simulink model "AmpelkreuzungV5_9"  (R2024b)
settings: Solver=FixedStepAuto  StartTime=0.0  StopTime=5000  FixedStep=1  RelTol=1e-3
model workspace (MATLAB code in the model file):
  | function [autos_l1, autos_rg1, autos_2l, autos_2rg, autos_3l, autos_3rg, autos_4, fehler] = generateCars(Auslastung)
  |     if (auslastung == 1)
  |         autos_l1 = round(randn());
  |         autos_rg1 = round(randn());
  |         autos_2l = round(randn());
  |         autos_2rg = round(randn());
  |         autos_3l = round(randn());
  |         autos_3rg = round(randn());
  |         autos_4 = round(randn());
  |     else
  |         fehler = 1;
  |     end
  | 
  |     if (auslastung == 2)
  |         autos_l1 = round(randn());
  |         autos_rg1 = round(4 + 2 * randn());
  |         autos_2l = round(1 + randn());
  |         autos_2rg = round(4 + 2 * randn());
  |         autos_3l = round(randn());
  |         autos_3rg = round(2 + randn());
  |         autos_4 = round(1 + randn());
  |     else
  |         fehler = 1;
  |     end
  | 
  |     if (auslastung == 3)
  |         autos_l1 = round(1.5 + randn());
  |         autos_rg1 = round(7 + 2 * randn());
  |         autos_2l = round(2 + randn());
  |         autos_2rg = round(7 + 2 * randn());
  |         autos_3l = round(2 * randn());
  |         autos_3rg = round(3 + randn());
  |         autos_4 = round(2 + randn());
  |     else
  |         fehler = 1;
  |     end
  | 
  |     if (auslastung == 4)
  |         autos_l1 = round(2.5 + randn());
  |         autos_rg1 = round(13 + 3 * randn());
  |         autos_2l = round(5 + randn());
  |         autos_2rg = round(13 + 3 * randn());
  |         autos_3l = round(2 + randn());
  |         autos_3rg = round(2 + randn());
  |         autos_4 = round(5 + randn());
  |     else
  |         fehler = 1;
  |     end
  | end
(part 2 of 3)

== stateflow chart AmpelkreuzungV5_9/Chart ==
  state Start
    entry:
    clear all;
    rot1_l = 1;
    gelb1_l = 0;
    gruen1_l = 0;
    rot1_rg = 1;
    gelb1_rg = 0;
    gruen1_rg = 0;
    rot2 = 1;
    gelb2 = 0;
    gruen2 = 0;
    rot3_l = 1;
    gelb3_l = 0;
    gruen3_l = 0;
    rot3_rg = 1;
    gelb3_rg = 0;
    gruen3_rg = 0;
    rot4 = 1;
    gelb4 = 0;
    gruen4 = 0;
    rot5 = 1;
    gruen5 = 0;
    rot6 = 1;
    gruen6 = 0;
    rot7 = 1;
    gruen7 = 0;
    rot8 = 1;
    gruen8 = 0;
    timeCounter = 0;
    timer_spuren = [0 0 0 0 0 0 0];
    gesamtZeit = 0;
    gesamte_autos = 0;
    %alle_autos = [0 0 0 0 0 0 0; 0 0 0 0 0 0 0];
    spur1 = zeros(1,N / 2);
    spur2 = zeros(1,N / 2);
    spur3 = zeros(1,N / 2);
    spur4 = zeros(1,N / 2);
    spur5 = zeros(1,N / 2);
    spur6 = zeros(1,N / 2);
    spur7 = zeros(1,N / 2);
    autos_auf_spur1 = 0;
    autos_auf_spur2 = 0;
    autos_auf_spur3 = 0;
    autos_auf_spur4 = 0;
    autos_auf_spur5 = 0;
    autos_auf_spur6 = 0;
    autos_auf_spur7 = 0;
    counter = [0 0 0 0 0 0 0];
    anz_autos1 = 0;
    anz_autos2 = 0;
    anz_autos3 = 0;
    anz_autos4 = 0;
    anz_autos5 = 0;
    anz_autos6 = 0;
    anz_autos7 = 0;
    wartezeit_spur1_ges = 0;
    wartezeit_spur2_ges = 0;
    wartezeit_spur3_ges = 0;
    wartezeit_spur4_ges = 0;
    wartezeit_spur5_ges = 0;
    wartezeit_spur6_ges = 0;
    wartezeit_spur7_ges = 0;
    krit1 = 0;
    krit2 = 0;
    krit3 = 0;
  state dokumentiere_startzeiten_initialisiere_wartezeiten
    en:
    startzeiten1 = spur1;
    startzeiten2 = spur2;
    startzeiten3 = spur3;
    startzeiten4 = spur4;
    startzeiten5 = spur5;
    startzeiten6 = spur6;
    startzeiten7 = spur7;
    wartezeiten1 = zeros(1, length(startzeiten1));
    wartezeiten2 = zeros(1, length(startzeiten2));
    wartezeiten3 = zeros(1, length(startzeiten3));
    wartezeiten4 = zeros(1, length(startzeiten4));
    wartezeiten5 = zeros(1, length(startzeiten5));
    wartezeiten6 = zeros(1, length(startzeiten6));
    wartezeiten7 = zeros(1, length(startzeiten7));
  state endzeiten_initialisieren
    en:
    endzeiten1 = zeros(1, length(spur1));
    endzeiten2 = zeros(1, length(spur2));
    endzeiten3 = zeros(1, length(spur3));
    endzeiten4 = zeros(1, length(spur4));
    endzeiten5 = zeros(1, length(spur5));
    endzeiten6 = zeros(1, length(spur6));
    endzeiten7 = zeros(1, length(spur7));
  state rg1_ampel2_rotgelb
    entry:
    gelb1_rg = 1;
    gelb2 = 1;
  state l1_rg1_rotgelb
    entry:
    gelb1_l = 1;
    gelb1_rg = 1;
  state rg1_ampel2_gruen
    entry:
    rot1_rg = 0;
    gelb1_rg = 0;
    gruen1_rg = 1;
    rot2 = 0;
    gelb2 = 0;
    gruen2 = 1;
    rot7 = 0;
    gruen7 = 1;
    rot8 = 0;
    gruen8 = 1;
  state l1_rg1_gruen
    entry:
    rot1_l = 0;
    gelb1_l = 0;
    gruen1_l = 1;
    rot1_rg = 0;
    gelb1_rg = 0;
    gruen1_rg = 1;
    rot7 = 0;
    gruen7 = 1;
  state rg1_ampel2_rotgelb1
    entry:
    gelb1_rg = 1;
    gelb2 = 1;
  state rg1_ampel2_rotgelb2
    entry:
    gelb1_rg = 1;
    gelb2 = 1;
  state l1_rg1_rotgelb1
    entry:
    gelb1_l = 1;
    gelb1_rg = 1;
  state l1_rg1_rotgelb2
    entry:
    gelb1_l = 1;
    gelb1_rg = 1;
  state l1_gelb
    entry:
    gelb1_l = 1;
    gruen1_l = 0;
  state rg1_ampel2_gruen1
    entry:
    rot1_rg = 0;
    gelb1_rg = 0;
    gruen1_rg = 1;
    rot2 = 0;
    gelb2 = 0;
    gruen2 = 1;
    rot7 = 0;
    gruen7 = 1;
    rot8 = 0;
    gruen8 = 1;
  state rg1_ampel2_gruen2
    entry:
    rot1_rg = 0;
    gelb1_rg = 0;
    gruen1_rg = 1;
    rot2 = 0;
    gelb2 = 0;
    gruen2 = 1;
    rot7 = 0;
    gruen7 = 1;
    rot8 = 0;
    gruen8 = 1;
  state l1_rg1_gruen1
    entry:
    rot1_l = 0;
    gelb1_l = 0;
    gruen1_l = 1;
    rot1_rg = 0;
    gelb1_rg = 0;
    gruen1_rg = 1;
    rot7 = 0;
    gruen7 = 1;
  state rg1_ampel2_rotgelb3
    entry:
    gelb1_rg = 1;
    gelb2 = 1;
  state l1_rg1_gruen2
    entry:
    rot1_l = 0;
    gelb1_l = 0;
    gruen1_l = 1;
    rot1_rg = 0;
    gelb1_rg = 0;
    gruen1_rg = 1;
    rot7 = 0;
    gruen7 = 1;
  state l1_rot
    entry:
    rot1_l = 1;
    gelb1_l = 0;
  state l1_rg1_rotgelb3
    entry:
    gelb1_l = 1;
    gelb1_rg = 1;
  state Fuss7_rot1
    entry:
    rot7 = 1;
    gruen7 = 0;
  state rg1_ampel2_gruen3
    entry:
    rot1_rg = 0;
    gelb1_rg = 0;
    gruen1_rg = 1;
    rot2 = 0;
    gelb2 = 0;
    gruen2 = 1;
    rot7 = 0;
    gruen7 = 1;
    rot8 = 0;
    gruen8 = 1;
  state l1_gelb1
    entry:
    gelb1_l = 1;
    gruen1_l = 0;
  state l1_gelb2
    entry:
    gelb1_l = 1;
    gruen1_l = 0;
  state l1_rg1_gruen3
    entry:
    rot1_l = 0;
    gelb1_l = 0;
    gruen1_l = 1;
    rot1_rg = 0;
    gelb1_rg = 0;
    gruen1_rg = 1;
    rot7 = 0;
    gruen7 = 1;
  state l1_rot1
    entry:
    rot1_l = 1;
    gelb1_l = 0;
  state rg1_gelb1
    entry:
    gelb1_rg = 1;
    gruen1_rg = 0;
  state l1_rot2
    entry:
    rot1_l = 1;
    gelb1_l = 0;
  state ampel2_rotgelb
    entry:
    gelb2 = 1;
  state l1_rot4
    entry:
    rot1_l = 1;
    gelb1_l = 0;
  state Fuss7_rot2
    entry:
    rot7 = 1;
    gruen7 = 0;
  state Fuss7_rot4
    entry:
    rot7 = 1;
    gruen7 = 0;
  state ampel2_fuss8_gruen
    rot2 = 0;
    gelb2 = 0;
    gruen2 = 1;
    rot8 = 0;
    gruen8 = 1;
  state l1_gelb3
    entry:
    gelb1_l = 1;
    gruen1_l = 0;
  state rg1_rot1
    entry:
    gelb1_rg = 0;
    rot1_rg = 1;
  state l1_rot3
    entry:
    rot1_l = 1;
    gelb1_l = 0;
  state rg1_gelb2
    entry:
    gelb1_rg = 1;
    gruen1_rg = 0;
  state l1_rot6
    entry:
    rot1_l = 1;
    gelb1_l = 0;
  state l1_rot5
    entry:
    rot1_l = 1;
    gelb1_l = 0;
  state rg1_gelb4
    entry:
    gelb1_rg = 1;
    gruen1_rg = 0;
  state Fuss7_rot6
    entry:
    rot7 = 1;
    gruen7 = 0;
  state ampel2_rotgelb1
    entry:
    gelb2 = 1;
  state ampel2_rotgelb2
    entry:
    gelb2 = 1;
  state ampel2_fuss8_gruen1
    rot2 = 0;
    gelb2 = 0;
    gruen2 = 1;
    rot8 = 0;
    gruen8 = 1;
  state Fuss7_rot
    entry:
    rot7 = 1;
    gruen7 = 0;
  state ampel2_fuss8_gruen2
    rot2 = 0;
    gelb2 = 0;
    gruen2 = 1;
    rot8 = 0;
    gruen8 = 1;
  state rg1_rot6
    entry:
    gelb1_rg = 0;
    rot1_rg = 1;
  state rg1_rot13
    entry:
    gelb1_rg = 0;
    rot1_rg = 1;
  state l1_rot7
    entry:
    rot1_l = 1;
    gelb1_l = 0;
  state rg1_gelb7
    entry:
    gelb1_rg = 1;
    gruen1_rg = 0;
  state rg1_gelb
    entry:
    gelb1_rg = 1;
    gruen1_rg = 0;
  state fuss7_rot
    entry:
    rot7 = 1;
    gruen7 = 0;
  state rg1_rot20
    entry:
    gelb1_rg = 0;
    rot1_rg = 1;
  state rg1_rot
    entry:
    gelb1_rg = 0;
    rot1_rg = 1;
  state Fuss7_rot3
    entry:
    rot7 = 1;
    gruen7 = 0;
  state Fuss7_rot5
    entry:
    rot7 = 1;
    gruen7 = 0;
  state rg1_rot5
    entry:
    gelb1_rg = 0;
    rot1_rg = 1;
  state ampel2_rotgelb3
    entry:
    gelb2 = 1;
  state rg1_gelb3
    entry:
    gelb1_rg = 1;
    gruen1_rg = 0;
  state rg1_gelb5
    entry:
    gelb1_rg = 1;
    gruen1_rg = 0;
  state ampel2_fuss8_gruen3
    rot2 = 0;
    gelb2 = 0;
    gruen2 = 1;
    rot8 = 0;
    gruen8 = 1;
  state rg1_rot7
    entry:
    gelb1_rg = 0;
    rot1_rg = 1;
  state rg1_rot14
    entry:
    gelb1_rg = 0;
    rot1_rg = 1;
  state rg1_rot4
    entry:
    gelb1_rg = 0;
    rot1_rg = 1;
  state rg1_gelb6
    entry:
    gelb1_rg = 1;
    gruen1_rg = 0;
  state rg1_rot11
    entry:
    gelb1_rg = 0;
    rot1_rg = 1;
  state fuss8_rot7
    entry:
    rot8 = 1;
    gruen8 = 0;
  state rg1_rot17
    entry:
    gelb1_rg = 0;
    rot1_rg = 1;
  state fuss8_rot11
    entry:
    rot8 = 1;
    gruen8 = 0;
  state rg1_rot9
    entry:
    gelb1_rg = 0;
    rot1_rg = 1;
  state rg1_rot12
    entry:
    gelb1_rg = 0;
    rot1_rg = 1;
  state fuss8_rot8
    entry:
    rot8 = 1;
    gruen8 = 0;
  state rg1_rot21
    entry:
    gelb1_rg = 0;
    rot1_rg = 1;
  state rg1_rot16
    entry:
    gelb1_rg = 0;
    rot1_rg = 1
  state fuss8_rot9
    entry:
    rot8 = 1;
    gruen8 = 0;
  state rg1_rot15
    entry:
    gelb1_rg = 0;
    rot1_rg = 1
  state fuss8_rot5
    entry:
    rot8 = 1;
    gruen8 = 0;
  state fuss8_rot4
    entry:
    rot8 = 1;
    gruen8 = 0;
  state rg1_rot19
    entry:
    gelb1_rg = 0;
    rot1_rg = 1
  state ampel2_gelb8
    entry:
    gelb2 = 1;
    gruen2 = 0;
  state rg1_rot3
    entry:
    gelb1_rg = 0;
    rot1_rg = 1
  state rg1_rot18
    entry:
    gelb1_rg = 0;
    rot1_rg = 1
  state ampel2_gelb6
    entry:
    gelb2 = 1;
    gruen2 = 0;
  state ampel2_gelb11
    entry:
    gelb2 = 1;
    gruen2 = 0;
  state ampel2_gelb7
    entry:
    gelb2 = 1;
    gruen2 = 0;
  state ampel2_gelb5
    entry:
    gelb2 = 1;
    gruen2 = 0;
  state rg1_rot2
    entry:
    gelb1_rg = 0;
    rot1_rg = 1
  state ampel2_gelb4
    entry:
    gelb2 = 1;
    gruen2 = 0;
  state fuss8_rot10
    entry:
    rot8 = 1;
    gruen8 = 0;
  state fuss8_rot12
    entry:
    rot8 = 1;
    gruen8 = 0;
  state fuss8_rot1
    entry:
    rot8 = 1;
    gruen8 = 0;
  state fuss8_rot
    entry:
    rot8 = 1;
    gruen8 = 0;
  state ampel2_rot12
    rot2 = 1;
    gelb2 = 0;
  state ampel2_gelb9
    entry:
    gelb2 = 1;
    gruen2 = 0;
  state ampel2_rot11
    rot2 = 1;
    gelb2 = 0;
  state ampel2_gelb10
    entry:
    gelb2 = 1;
    gruen2 = 0;
  state ampel2_gelb1
    entry:
    gelb2 = 1;
    gruen2 = 0;
  state rg1_rot8
    entry:
    gelb1_rg = 0;
    rot1_rg = 1
  state ampel2_gelb
    entry:
    gelb2 = 1;
    gruen2 = 0;
  state rg1_rot10
    entry:
    gelb1_rg = 0;
    rot1_rg = 1
  state ampel2_rot13
    rot2 = 1;
    gelb2 = 0;
  state fuss8_rot3
    entry:
    rot8 = 1;
    gruen8 = 0;
  state ampel2_rot9
    rot2 = 1;
    gelb2 = 0;
  state ampel2_rot19
    rot2 = 1;
    gelb2 = 0;
  state fuss8_rot2
    entry:
    rot8 = 1;
    gruen8 = 0;
  state ampel2_rot17
    rot2 = 1;
    gelb2 = 0;
  state ampel2_rot
    rot2 = 1;
    gelb2 = 0;
  state ampel2_gelb3
    entry:
    gelb2 = 1;
    gruen2 = 0;
  state ampel2_gelb2
    entry:
    gelb2 = 1;
    gruen2 = 0;
  state ampel2_rot21
    rot2 = 1;
    gelb2 = 0;
  state ampel2_rot20
    rot2 = 1;
    gelb2 = 0;
  state ampel2_rot1
    rot2 = 1;
    gelb2 = 0;
  state ampel2_rot5
    rot2 = 1;
    gelb2 = 0;
  state ampel2_rot14
    rot2 = 1;
    gelb2 = 0;
  state ampel2_rot10
    rot2 = 1;
    gelb2 = 0;
  state ampel2_rot6
    rot2 = 1;
    gelb2 = 0;
  state ampel2_rot15
    rot2 = 1;
    gelb2 = 0;
  state ampel2_rot8
    rot2 = 1;
    gelb2 = 0;
  state rg3_rotgelb7
    entry:
    gelb3_rg = 1;
  state rg3_rotgelb4
    entry:
    gelb3_rg = 1;
  state rg3_rotgelb8
    entry:
    gelb3_rg = 1;
  state rg3_rotgelb5
    entry:
    gelb3_rg = 1;
  state ampel2_rot16
    rot2 = 1;
    gelb2 = 0;
  state ampel2_rot22
    rot2 = 1;
    gelb2 = 0;
  state ampel2_rot18
    rot2 = 1;
    gelb2 = 0;
  state ampel2_rot2
    rot2 = 1;
    gelb2 = 0;
  state ampel2_rot23
    rot2 = 1;
    gelb2 = 0;
  state ampel2_rot3
    rot2 = 1;
    gelb2 = 0;
  state rg3_rotgelb10
    entry:
    gelb3_rg = 1;
  state rg3_rotgelb11
    entry:
    gelb3_rg = 1;
  state rg3_rotgelb12
    entry:
    gelb3_rg = 1;
  state rg3_rotgelb
    entry:
    gelb3_rg = 1;
  state rg3_rotgelb9
    entry:
    gelb3_rg = 1;
  state rg3_rotgelb1
    entry:
    gelb3_rg = 1;
  state ampel2_rot7
    rot2 = 1;
    gelb2 = 0;
  state ampel2_rot4
    rot2 = 1;
    gelb2 = 0;
  state rg3_rotgelb2
    entry:
    gelb3_rg = 1;
  state l3_rotgelb_rg3_fuss6_gruen
    entry:
    gelb3_l = 1;
    rot3_rg = 0;
    gelb3_rg = 0;
    gruen3_rg = 1;
    rot6 = 0;
    gruen6 = 1;
  state rg3_fuss6_gruen
    entry:
    rot3_rg = 0;
    gelb3_rg = 0;
    gruen3_rg = 1;
    rot6 = 0;
    gruen6 = 1;
  state rg3_rotgelb3
    entry:
    gelb3_rg = 1;
  state ampel4_rotgelb
    entry:
    gelb4 = 1;
  state rg3_rotgelb6
    entry:
    gelb3_rg = 1;
  state l3_gruen
    entry:
    rot3_l = 0;
    gelb3_l = 0;
    gruen3_l = 1;
  state l3_rotgelb_rg3_fuss6_gruen1
    entry:
    gelb3_l = 1;
    rot3_rg = 0;
    gelb3_rg = 0;
    gruen3_rg = 1;
    rot6 = 0;
    gruen6 = 1;
  state rg3_fuss6_gruen1
    entry:
    rot3_rg = 0;
    gelb3_rg = 0;
    gruen3_rg = 1;
    rot6 = 0;
    gruen6 = 1;
  state l3_rotgelb_rg3_fuss6_gruen2
    entry:
    gelb3_l = 1;
    rot3_rg = 0;
    gelb3_rg = 0;
    gruen3_rg = 1;
    rot6 = 0;
    gruen6 = 1;
  state rg3_fuss6_gruen2
    entry:
    rot3_rg = 0;
    gelb3_rg = 0;
    gruen3_rg = 1;
    rot6 = 0;
    gruen6 = 1;
  state l3_gelb
    entry:
    gelb3_l = 1;
    gruen3_l = 0;
  state ampel4_rotgelb1
    entry:
    gelb4 = 1;
  state ampel4_rotgelb2
    entry:
    gelb4 = 1;
  state l3_gruen1
    entry:
    rot3_l = 0;
    gelb3_l = 0;
    gruen3_l = 1;
  state ampel4_fuss5_gruen
    entry:
    rot4 = 0;
    gelb4 = 0;
    gruen4 = 1;
    rot5 = 0;
    gruen5 = 1;
  state l3_rotgelb_rg3_fuss6_gruen3
    entry:
    gelb3_l = 1;
    rot3_rg = 0;
    gelb3_rg = 0;
    gruen3_rg = 1;
    rot6 = 0;
    gruen6 = 1;
  state rg3_fuss6_gruen3
    entry:
    rot3_rg = 0;
    gelb3_rg = 0;
    gruen3_rg = 1;
    rot6 = 0;
    gruen6 = 1;
  state l3_gruen2
    entry:
    rot3_l = 0;
    gelb3_l = 0;
    gruen3_l = 1;
  state l3_fuss6_rot
    entry:
    rot3_l = 1;
    gelb3_l = 0;
    rot6 = 1;
    gruen6 = 0;
  state ampel4_rotgelb3
    entry:
    gelb4 = 1;
  state l3_gelb_fuss6_rot
    entry:
    gelb3_l = 1;
    gruen3_l = 0;
  state l3_gelb1
    entry:
    gelb3_l = 1;
    gruen3_l = 0;
  state l3_gruen3
    entry:
    rot3_l = 0;
    gelb3_l = 0;
    gruen3_l = 1;
  state ampel4_fuss5_gruen2
    entry:
    rot4 = 0;
    gelb4 = 0;
    gruen4 = 1;
    rot5 = 0;
    gruen5 = 1;
  state ampel4_fuss5_gruen4
    entry:
    rot4 = 0;
    gelb4 = 0;
    gruen4 = 1;
    rot5 = 0;
    gruen5 = 1;
  state fuss6_rot2
    entry:
    rot6 = 1;
    gruen6 = 0;
  state l3_fuss6_rot3
    entry:
    rot3_l = 1;
    gelb3_l = 0;
    rot6 = 1;
    gruen6 = 0;
  state l3_gelb2
    entry:
    gelb3_l = 1;
    gruen3_l = 0;
  state l3_fuss6_rot1
    entry:
    rot3_l = 1;
    gelb3_l = 0;
    rot6 = 1;
    gruen6 = 0;
  state l3_rot1
    entry:
    rot3_l = 1;
    gelb3_l = 0;
  state ampel4_fuss5_gruen6
    entry:
    rot4 = 0;
    gelb4 = 0;
    gruen4 = 1;
    rot5 = 0;
    gruen5 = 1;
  state fuss6_rot
    entry:
    rot6 = 1;
    gruen6 = 0;
  state fuss6_rot4
    entry:
    rot6 = 1;
    gruen6 = 0;
  state rg3_gelb1
    entry:
    gelb3_rg = 1;
    gruen3_rg = 0;
  state rg3_gelb
    entry:
    gelb3_rg = 1;
    gruen3_rg = 0;
  state l3_rot_rg3_gelb
    entry:
    rot3_l = 1;
    gelb3_l = 0;
    gelb3_rg = 1;
    gruen3_rg = 0;
  state l3_fuss6_rot2
    entry:
    rot3_l = 1;
    gelb3_l = 0;
    rot6 = 1;
    gruen6 = 0;
  state l3_rot
    entry:
    rot3_l = 1;
    gelb3_l = 0;
  state fuss6_rot1
    entry:
    rot6 = 1;
    gruen6 = 0;
  state fuss6_rot3
    entry:
    rot6 = 1;
    gruen6 = 0;
  state rg3_rot_ampel4_rotgelb
    entry:
    rot3_rg = 1;
    gelb3_rg = 0;
    gelb4 = 1;
  state rg3_gelb2
    entry:
    gelb3_rg = 1;
    gruen3_rg = 0;
  state rg3_gelb3
    entry:
    gelb3_rg = 1;
    gruen3_rg = 0;
  state rg3_gelb4
    entry:
    gelb3_rg = 1;
    gruen3_rg = 0;
  state rg3_gelb5
    entry:
    gelb3_rg = 1;
    gruen3_rg = 0;
  state rg3_fuss5_rot
    entry:
    rot3_rg = 1;
    gelb3_rg = 0;
    rot5 = 1;
    gruen5 = 0;
  state fuss6_rot5
    entry:
    rot6 = 1;
    gruen6 = 0;
  state l3_rot_rg3_gelb1
    entry:
    rot3_l = 1;
    gelb3_l = 0;
    gelb3_rg = 1;
    gruen3_rg = 0;
  state rg3_gelb6
    entry:
    gelb3_rg = 1;
    gruen3_rg = 0;
  state rg3_rot_ampel4_rotgelb2
    entry:
    rot3_rg = 1;
    gelb3_rg = 0;
    gelb4 = 1;
  state rg3_rot_ampel4_rotgelb4
    entry:
    rot3_rg = 1;
    gelb3_rg = 0;
    gelb4 = 1;
  state rg3_rot_ampel4_rotgelb1
    entry:
    rot3_rg = 1;
    gelb3_rg = 0;
    gelb4 = 1;
  state rg3_fuss5_rot2
    entry:
    rot3_rg = 1;
    gelb3_rg = 0;
    rot5 = 1;
    gruen5 = 0;
  state rg3_fuss5_rot5
    entry:
    rot3_rg = 1;
    gelb3_rg = 0;
    rot5 = 1;
    gruen5 = 0;
  state rg3_rot_ampel4_rotgelb6
    entry:
    rot3_rg = 1;
    gelb3_rg = 0;
    gelb4 = 1;
  state ampel4_fuss5_gruen1
    entry:
    rot4 = 0;
    gelb4 = 0;
    gruen4 = 1;
    rot5 = 0;
    gruen5 = 1;
  state rg3_fuss5_rot6
    entry:
    rot3_rg = 1;
    gelb3_rg = 0;
    rot5 = 1;
    gruen5 = 0;
  state rg3_rot_ampel4_rotgelb3
    entry:
    rot3_rg = 1;
    gelb3_rg = 0;
    gelb4 = 1;
  state rg3_rot_ampel4_rotgelb5
    entry:
    rot3_rg = 1;
    gelb3_rg = 0;
    gelb4 = 1;
  state fuss5_rot
    entry:
    rot5 = 1;
    gruen5 = 0;
  state ampel4_fuss5_gruen3
    entry:
    rot4 = 0;
    gelb4 = 0;
    gruen4 = 1;
    rot5 = 0;
    gruen5 = 1;
  state ampel4_fuss5_gruen5
    entry:
    rot4 = 0;
    gelb4 = 0;
    gruen4 = 1;
    rot5 = 0;
    gruen5 = 1;
  state rg3_rot_ampel4_rotgelb7
    entry:
    rot3_rg = 1;
    gelb3_rg = 0;
    gelb4 = 1;
  state rg3_fuss5_rot1
    entry:
    rot3_rg = 1;
    gelb3_rg = 0;
    rot5 = 1;
    gruen5 = 0;
  state ampel4_fuss5_gruen7
    entry:
    rot4 = 0;
    gelb4 = 0;
    gruen4 = 1;
    rot5 = 0;
    gruen5 = 1;
  state fuss5_rot1
    entry:
    rot5 = 1;
    gruen5 = 0;
  state fuss5_rot2
    entry:
    rot5 = 1;
    gruen5 = 0;
  state rg3_fuss5_rot3
    entry:
    rot3_rg = 1;
    gelb3_rg = 0;
    rot5 = 1;
    gruen5 = 0;
  state rg3_fuss5_rot4
    entry:
    rot3_rg = 1;
    gelb3_rg = 0;
    rot5 = 1;
    gruen5 = 0;
  state fuss5_rot3
    entry:
    rot5 = 1;
    gruen5 = 0;
  state ampel4_gelb
    entry:
    gelb4 = 1;
    gruen4 = 0;
  state rg3_fuss5_rot7
    entry:
    rot3_rg = 1;
    gelb3_rg = 0;
    rot5 = 1;
    gruen5 = 0;
  state ampel4_rot
    entry:
    rot4 = 1;
    gelb4 = 0;
  state ampel4_rot2
    entry:
    rot4 = 1;
    gelb4 = 0;
  state ampel4_gelb1
    entry:
    gelb4 = 1;
    gruen4 = 0;
  state ampel4_gelb2
    entry:
    gelb4 = 1;
    gruen4 = 0;
  state ampel4_rot3
    entry:
    rot4 = 1;
    gelb4 = 0;
  state ampel4_rot5
    entry:
    rot4 = 1;
    gelb4 = 0;
  state ampel4_gelb3
    entry:
    gelb4 = 1;
    gruen4 = 0;
  state ampel4_rot4
    entry:
    rot4 = 1;
    gelb4 = 0;
  state ampel4_rot6
    entry:
    rot4 = 1;
    gelb4 = 0;
  state ampel4_rot7
    entry:
    rot4 = 1;
    gelb4 = 0;
  state ampel4_rot8
    entry:
    rot4 = 1;
    gelb4 = 0;
  (default) -> Start
  Start -> (junction 796) : {zeit_abstand = zeit_abstand_aus_auslastung(auslastung);}
  (junction 796) -> (junction 748) : {alle_autos_neu  = generiere_autos_neu(N, zeit_abstand, auslastung);}
  (junction 748) -> dokumentiere_startzeiten_initialisiere_wartezeiten : {[spur1, spur2, spur3, spur4, spur5, spur6, spur7] = spuren_aus_autos(alle_autos_neu, N);}
  dokumentiere_startzeiten_initialisiere_wartezeiten -> endzeiten_initialisieren
  endzeiten_initialisieren -> (junction 248)
  (junction 181) -> (junction 248) : {timeCounter = resetTimer()}
  (junction 248) -> (junction 1426) [order 1] : [auslastung == 5]
  (junction 248) -> (junction 1428) [order 2]
  (junction 179) -> (junction 181)
  (junction 1426) -> (junction 1092) : {alte_counter = counter;}
  (junction 1428) -> (junction 1430) [order 1] : [auslastung == 4]
  (junction 1428) -> (junction 1840) [order 2]
  (junction 1430) -> (junction 1670) : {alte_counter = counter;}
  (junction 1840) -> (junction 1843) [order 1] : [auslastung == 3]
  (junction 1840) -> (junction 3331) [order 2]
  (junction 1843) -> (junction 2751) : {alte_counter = counter;}
  (junction 3331) -> (junction 3333) : [auslastung == 1 || auslastung == 2]
  (junction 3333) -> (junction 3239) : {alte_counter = counter;}
  (junction 1092) -> (junction 1075) : after(1,sec)
      | {timeCounter = refresher(timeCounter, 1);}
  (junction 1075) -> (junction 1077) : {timer_spuren = countOnwards(timer_spuren,1,[1 1 1 1 1 1 1]);}
      |
      | %Linksabbieger1
  (junction 1077) -> (junction 1076) : {[autos_auf_spur1, spur1] = autos_auf_spur_generieren(spur1, gesamtZeit + timeCounter + 2, autos_auf_spur1);}
  (junction 1076) -> (junction 1081) : {autos_spur1_flag = false;}
  (junction 1670) -> (junction 1696) : after(1,sec)
      | {timeCounter = refresher(timeCounter, 1);}
  (junction 2751) -> (junction 2752) : after(1,sec)
      | {timeCounter = refresher(timeCounter, 1);}
  (junction 1081) -> (junction 1085) [order 1] : [autos_auf_spur1 == 0]
  (junction 1696) -> (junction 1673) : {timer_spuren = countOnwards(timer_spuren,1,[1 1 1 1 1 1 1]);}
      |
      | %Linksabbieger1
  (junction 1081) -> (junction 1084) [order 2]
  (junction 1085) -> rg1_ampel2_rotgelb
  (junction 2752) -> (junction 2755) : {timer_spuren = countOnwards(timer_spuren,1,[1 1 1 1 1 1 1]);}
      |
      | %Linksabbieger1
  (junction 1084) -> (junction 1074) [order 1] : [autos_auf_spur1 > 0]
  (junction 1084) -> (junction 1111) [order 2]
  (junction 1074) -> l1_rg1_rotgelb : {autos_spur1_flag = true;}
  rg1_ampel2_rotgelb -> (junction 1097) : after(1,sec)
      | {timeCounter = refresher(timeCounter, 1);}
  (junction 1673) -> (junction 1668) : {[autos_auf_spur1, spur1] = autos_auf_spur_generieren(spur1, gesamtZeit + timeCounter + 2, autos_auf_spur1);}
  (junction 2755) -> (junction 2748) : {[autos_auf_spur1, spur1] = autos_auf_spur_generieren(spur1, gesamtZeit + timeCounter + 2, autos_auf_spur1);}
  (junction 1097) -> rg1_ampel2_gruen : {timer_spuren = countOnwards(timer_spuren,1,[1 1 1 1 1 1 1]);}
  l1_rg1_rotgelb -> (junction 1082) : after(1,sec)
      | {timeCounter = refresher(timeCounter, 1);}
  (junction 1082) -> l1_rg1_gruen : {timer_spuren = countOnwards(timer_spuren,1,[1 1 1 1 1 1 1]);}
  (junction 3239) -> (junction 3238) : after(1,sec)
      | {timeCounter = refresher(timeCounter, 1);}
  (junction 1668) -> (junction 1687) : {autos_spur1_flag = false;}
  (junction 2748) -> (junction 2753) : {autos_spur1_flag = false;}
  (junction 3238) -> (junction 3241) : {timer_spuren = countOnwards(timer_spuren,1,[1 1 1 1 1 1 1]);}
      |
      | %Linksabbieger1
  rg1_ampel2_gruen -> (junction 1080) : {[autos_auf_spur2, spur2] = autos_auf_spur_generieren(spur2, gesamtZeit + timeCounter, autos_auf_spur2);}
  (junction 1687) -> (junction 1688) [order 1] : [autos_auf_spur1 == 0]
  (junction 1687) -> (junction 1690) [order 2]
  (junction 1688) -> rg1_ampel2_rotgelb1
  (junction 3241) -> (junction 3240) : {[autos_auf_spur1, spur1] = autos_auf_spur_generieren(spur1, gesamtZeit + timeCounter + 2, autos_auf_spur1);}
  (junction 2753) -> (junction 2754) [order 1] : [autos_auf_spur1 == 0]
  (junction 2754) -> rg1_ampel2_rotgelb2
  (junction 2753) -> (junction 2740) [order 2]
  (junction 1080) -> (junction 1098) : {[autos_auf_spur3, spur3] = autos_auf_spur_generieren(spur3, gesamtZeit + timeCounter, autos_auf_spur3);}
  l1_rg1_gruen -> (junction 1083) : {[autos_auf_spur1, spur1] = autos_auf_spur_generieren(spur1, gesamtZeit + timeCounter, autos_auf_spur1);}
  (junction 1690) -> (junction 1697) [order 1] : [autos_auf_spur1 > 0]
  (junction 1690) -> (junction 1741) [order 2]
  (junction 1697) -> l1_rg1_rotgelb1 : {autos_spur1_flag = true;}
  rg1_ampel2_rotgelb1 -> (junction 1698) : after(1,sec)
      | {timeCounter = refresher(timeCounter, 1);}
  (junction 2740) -> (junction 2746) [order 1] : [autos_auf_spur1 > 0]
  (junction 2740) -> (junction 2786) [order 2]
  (junction 2746) -> l1_rg1_rotgelb2 : {autos_spur1_flag = true;}
  rg1_ampel2_rotgelb2 -> (junction 2747) : after(1,sec)
      | {timeCounter = refresher(timeCounter, 1);}
  (junction 1083) -> (junction 1078) : {[autos_auf_spur2, spur2] = autos_auf_spur_generieren(spur2, gesamtZeit + timeCounter, autos_auf_spur2);}
  (junction 1098) -> (junction 1086) : {[autos_auf_spur4, spur4] = autos_auf_spur_generieren(spur4, gesamtZeit + timeCounter, autos_auf_spur4);}
  (junction 1078) -> (junction 1073) : after(8,sec)
      | {timeCounter = refresher(timeCounter, 8);}
  (junction 1698) -> rg1_ampel2_gruen1 : {timer_spuren = countOnwards(timer_spuren,1,[1 1 1 1 1 1 1]);}
  (junction 2747) -> rg1_ampel2_gruen2 : {timer_spuren = countOnwards(timer_spuren,1,[1 1 1 1 1 1 1]);}
  l1_rg1_rotgelb1 -> (junction 1715) : after(1,sec)
      | {timeCounter = refresher(timeCounter, 1);}
  (junction 3240) -> (junction 3243) : {autos_spur1_flag = false;}
  (junction 1073) -> l1_gelb : {timer_spuren = countOnwards(timer_spuren,8,[0 0 1 1 1 1 1]);}
  (junction 1086) -> (junction 1087) : after(45,sec)
      | {timeCounter = refresher(timeCounter, 45);}
  l1_rg1_rotgelb2 -> (junction 2742) : after(1,sec)
      | {timeCounter = refresher(timeCounter, 1);}
  (junction 1715) -> l1_rg1_gruen1 : {timer_spuren = countOnwards(timer_spuren,1,[1 1 1 1 1 1 1]);}
  (junction 2742) -> l1_rg1_gruen2 : {timer_spuren = countOnwards(timer_spuren,1,[1 1 1 1 1 1 1]);}
  l1_gelb -> (junction 1093) : after(3,sec)
      | {timeCounter = refresher(timeCounter, 3);}
  (junction 1087) -> Fuss7_rot1 : {timer_spuren = countOnwards(timer_spuren,45,[1 0 0 0 1 1 1]);}
  (junction 1093) -> (junction 1079) : {[autos_auf_spur1, spur1] = autos_auf_spur_generieren(spur1, gesamtZeit + timeCounter, autos_auf_spur1);}
  (junction 3243) -> (junction 3249) [order 1] : [autos_auf_spur1 == 0]
  (junction 3243) -> (junction 3244) [order 2]
  (junction 3249) -> rg1_ampel2_rotgelb3
  (junction 1079) -> l1_rot : {timer_spuren = countOnwards(timer_spuren,3,[0 0 1 1 1 1 1]);}
  (junction 3244) -> (junction 3245) [order 1] : [autos_auf_spur1 > 0]
  rg1_ampel2_gruen1 -> (junction 1704) : {[autos_auf_spur2, spur2] = autos_auf_spur_generieren(spur2, gesamtZeit + timeCounter, autos_auf_spur2);}
  (junction 3244) -> (junction 3120) [order 2]
  (junction 3245) -> l1_rg1_rotgelb3 : {autos_spur1_flag = true;}
  rg1_ampel2_gruen2 -> (junction 2749) : {[autos_auf_spur2, spur2] = autos_auf_spur_generieren(spur2, gesamtZeit + timeCounter, autos_auf_spur2);}
  rg1_ampel2_rotgelb3 -> (junction 3246) : after(1,sec)
      | {timeCounter = refresher(timeCounter, 1);}
  l1_rot -> (junction 1095) : {[anz_autos1, autos_auf_spur1, counter(1), endzeiten1] = generiere_gruenphase(1, 11, autos_auf_spur1, counter(1),  (gesamtZeit + timeCounter - 11), endzeiten1, startzeiten1, auslastung, autos_spur1_flag);}
  (junction 1704) -> (junction 1722) : {[autos_auf_spur3, spur3] = autos_auf_spur_generieren(spur3, gesamtZeit + timeCounter, autos_auf_spur3);}
  (junction 2749) -> (junction 2743) : {[autos_auf_spur3, spur3] = autos_auf_spur_generieren(spur3, gesamtZeit + timeCounter, autos_auf_spur3);}
  l1_rg1_gruen1 -> (junction 1720) : {[autos_auf_spur1, spur1] = autos_auf_spur_generieren(spur1, gesamtZeit + timeCounter, autos_auf_spur1);}
  (junction 3246) -> rg1_ampel2_gruen3 : {timer_spuren = countOnwards(timer_spuren,1,[1 1 1 1 1 1 1]);}
  (junction 1095) -> (junction 1096) : {wartezeiten1 = berechne_wartezeiten(startzeiten1, endzeiten1, alte_counter(1), counter(1), wartezeiten1);}
  l1_rg1_gruen2 -> (junction 2741) : {[autos_auf_spur1, spur1] = autos_auf_spur_generieren(spur1, gesamtZeit + timeCounter, autos_auf_spur1);}
  l1_rg1_rotgelb3 -> (junction 3247) : after(1,sec)
      | {timeCounter = refresher(timeCounter, 1);}
  (junction 1720) -> (junction 1711) : {[autos_auf_spur2, spur2] = autos_auf_spur_generieren(spur2, gesamtZeit + timeCounter, autos_auf_spur2);}
  (junction 1722) -> (junction 1712) : {[autos_auf_spur4, spur4] = autos_auf_spur_generieren(spur4, gesamtZeit + timeCounter, autos_auf_spur4);}
  (junction 2741) -> (junction 2744) : {[autos_auf_spur2, spur2] = autos_auf_spur_generieren(spur2, gesamtZeit + timeCounter, autos_auf_spur2);}
  (junction 2743) -> (junction 2750) : {[autos_auf_spur4, spur4] = autos_auf_spur_generieren(spur4, gesamtZeit + timeCounter, autos_auf_spur4);}
  (junction 1096) -> (junction 1099) : {wartezeit_spur1_ges = gesamt_wartezeit_pro_spur(wartezeiten1, wartezeit_spur1_ges, alte_counter(1), counter(1));}
  Fuss7_rot1 -> (junction 1072) : after(2,sec)
      | {timeCounter = refresher(timeCounter, 2);}
  (junction 3247) -> l1_rg1_gruen3 : {timer_spuren = countOnwards(timer_spuren,1,[1 1 1 1 1 1 1]);}
  (junction 1711) -> (junction 1721) : after(8,sec)
      | {timeCounter = refresher(timeCounter, 8);}
  (junction 2744) -> (junction 2745) : after(8,sec)
      | {timeCounter = refresher(timeCounter, 8);}
  (junction 1099) -> (junction 1090) : {gesamtwartezeit = berechne_gesamtwartezeit(wartezeit_spur1_ges, wartezeit_spur2_ges, wartezeit_spur3_ges, wartezeit_spur4_ges, wartezeit_spur5_ges, wartezeit_spur6_ges, wartezeit_spur7_ges);}
  (junction 1721) -> l1_gelb1 : {timer_spuren = countOnwards(timer_spuren,8,[0 0 1 1 1 1 1]);}
  (junction 1712) -> (junction 1723) : after(35,sec)
      | {timeCounter = refresher(timeCounter, 35);}
  (junction 2750) -> (junction 2758) : after(20,sec)
      | {timeCounter = refresher(timeCounter, 20);}
  (junction 2745) -> l1_gelb2 : {timer_spuren = countOnwards(timer_spuren,8,[0 0 1 1 1 1 1]);}
  (junction 1072) -> rg1_gelb1 : {timer_spuren = countOnwards(timer_spuren,2,[1 0 0 0 1 1 1]);}
  (junction 1090) -> l1_rot1 : {gesamte_autos = berechne_gesamte_autos(counter(1), counter(2), counter(3), counter(4), counter(5), counter(6), counter(7));}
  l1_gelb1 -> (junction 1724) : after(3,sec)
      | {timeCounter = refresher(timeCounter, 3);}
  (junction 1723) -> Fuss7_rot2 : {timer_spuren = countOnwards(timer_spuren,35,[1 0 0 0 1 1 1]);}
  (junction 2758) -> Fuss7_rot4 : {timer_spuren = countOnwards(timer_spuren,20,[1 0 0 0 1 1 1]);}
  l1_gelb2 -> (junction 2756) : after(3,sec)
      | {timeCounter = refresher(timeCounter, 3);}
  rg1_ampel2_gruen3 -> (junction 3242) : {[autos_auf_spur2, spur2] = autos_auf_spur_generieren(spur2, gesamtZeit + timeCounter, autos_auf_spur2);}
  (junction 1724) -> (junction 1719) : {[autos_auf_spur1, spur1] = autos_auf_spur_generieren(spur1, gesamtZeit + timeCounter, autos_auf_spur1);}
  l1_rot1 -> (junction 1088) : after(3,sec)
      | {timeCounter = refresher(timeCounter, 3);}
  (junction 2756) -> (junction 2757) : {[autos_auf_spur1, spur1] = autos_auf_spur_generieren(spur1, gesamtZeit + timeCounter, autos_auf_spur1);}
  rg1_gelb1 -> (junction 1089) : after(3,sec)
      | {timeCounter = refresher(timeCounter, 3);}
  (junction 1088) -> ampel2_rotgelb : {timer_spuren = countOnwards(timer_spuren,3,[1 0 1 1 1 1 1]);}
  (junction 3242) -> (junction 3258) : {[autos_auf_spur3, spur3] = autos_auf_spur_generieren(spur3, gesamtZeit + timeCounter, autos_auf_spur3);}
  (junction 1719) -> l1_rot2 : {timer_spuren = countOnwards(timer_spuren,3,[0 0 1 1 1 1 1]);}
  l1_rg1_gruen3 -> (junction 3248) : {[autos_auf_spur1, spur1] = autos_auf_spur_generieren(spur1, gesamtZeit + timeCounter, autos_auf_spur1);}
  (junction 2757) -> l1_rot4 : {timer_spuren = countOnwards(timer_spuren,3,[0 0 1 1 1 1 1]);}
  (junction 3248) -> (junction 3259) : {[autos_auf_spur2, spur2] = autos_auf_spur_generieren(spur2, gesamtZeit + timeCounter, autos_auf_spur2);}
  (junction 1089) -> (junction 1094) : {[autos_auf_spur2, spur2] = autos_auf_spur_generieren(spur2, gesamtZeit + timeCounter, autos_auf_spur2);}
  (junction 3258) -> (junction 3264) : {[autos_auf_spur4, spur4] = autos_auf_spur_generieren(spur4, gesamtZeit + timeCounter, autos_auf_spur4);}
  l1_rot2 -> (junction 1725) : {[anz_autos1, autos_auf_spur1, counter(1), endzeiten1] = generiere_gruenphase(1, 11, autos_auf_spur1, counter(1),  (gesamtZeit + timeCounter - 11), endzeiten1, startzeiten1, auslastung, autos_spur1_flag);}
  ampel2_rotgelb -> (junction 1091) : after(1,sec)
      | {timeCounter = refresher(timeCounter, 1);}
  l1_rot4 -> (junction 2759) : {[anz_autos1, autos_auf_spur1, counter(1), endzeiten1] = generiere_gruenphase(1, 11, autos_auf_spur1, counter(1),  (gesamtZeit + timeCounter - 11), endzeiten1, startzeiten1, auslastung, autos_spur1_flag);}
  (junction 3259) -> (junction 3265) : after(3,sec)
      | {timeCounter = refresher(timeCounter, 3);}
  (junction 1091) -> ampel2_fuss8_gruen : {timer_spuren = countOnwards(timer_spuren,1,[1 0 1 1 1 1 1]);}
  (junction 1725) -> (junction 1708) : {wartezeiten1 = berechne_wartezeiten(startzeiten1, endzeiten1, alte_counter(1), counter(1), wartezeiten1);}
  (junction 1094) -> rg1_rot1 : {timer_spuren = countOnwards(timer_spuren,3,[1 0 0 0 1 1 1]);}
  (junction 3265) -> l1_gelb3 : {timer_spuren = countOnwards(timer_spuren,3,[0 0 1 1 1 1 1]);}
  (junction 3264) -> (junction 3267) : after(5,sec)
      | {timeCounter = refresher(timeCounter, 5);}
  (junction 2759) -> (junction 2760) : {wartezeiten1 = berechne_wartezeiten(startzeiten1, endzeiten1, alte_counter(1), counter(1), wartezeiten1);}
  (junction 1708) -> (junction 1731) : {wartezeit_spur1_ges = gesamt_wartezeit_pro_spur(wartezeiten1, wartezeit_spur1_ges, alte_counter(1), counter(1));}
  Fuss7_rot2 -> (junction 1726) : after(2,sec)
      | {timeCounter = refresher(timeCounter, 2);}
  Fuss7_rot4 -> (junction 2762) : after(2,sec)
      | {timeCounter = refresher(timeCounter, 2);}
  (junction 2760) -> (junction 2761) : {wartezeit_spur1_ges = gesamt_wartezeit_pro_spur(wartezeiten1, wartezeit_spur1_ges, alte_counter(1), counter(1));}
  l1_gelb3 -> (junction 3260) : after(3,sec)
      | {timeCounter = refresher(timeCounter, 3);}
  (junction 3267) -> Fuss7_rot6 : {timer_spuren = countOnwards(timer_spuren,5,[1 0 0 0 1 1 1]);}
  (junction 1731) -> (junction 1727) : {gesamtwartezeit = berechne_gesamtwartezeit(wartezeit_spur1_ges, wartezeit_spur2_ges, wartezeit_spur3_ges, wartezeit_spur4_ges, wartezeit_spur5_ges, wartezeit_spur6_ges, wartezeit_spur7_ges);}
  ampel2_fuss8_gruen -> (junction 1107) : {[autos_auf_spur3, spur3] = autos_auf_spur_generieren(spur3, gesamtZeit + timeCounter, autos_auf_spur3);}
  rg1_rot1 -> (junction 1124) : {[anz_autos2, autos_auf_spur2, counter(2), endzeiten2] = generiere_gruenphase(2, 50, autos_auf_spur2, counter(2),  (gesamtZeit + timeCounter - 50), endzeiten2, startzeiten2, auslastung, autos_spur1_flag);}
  (junction 2761) -> (junction 2765) : {gesamtwartezeit = berechne_gesamtwartezeit(wartezeit_spur1_ges, wartezeit_spur2_ges, wartezeit_spur3_ges, wartezeit_spur4_ges, wartezeit_spur5_ges, wartezeit_spur6_ges, wartezeit_spur7_ges);}
  (junction 3260) -> (junction 3250) : {[autos_auf_spur1, spur1] = autos_auf_spur_generieren(spur1, gesamtZeit + timeCounter, autos_auf_spur1);}
  (junction 1726) -> rg1_gelb2 : {timer_spuren = countOnwards(timer_spuren,2,[1 0 0 0 1 1 1]);}
  (junction 1727) -> l1_rot3 : {gesamte_autos = berechne_gesamte_autos(counter(1), counter(2), counter(3), counter(4), counter(5), counter(6), counter(7));}
  (junction 2762) -> rg1_gelb4 : {timer_spuren = countOnwards(timer_spuren,2,[1 0 0 0 1 1 1]);}
  (junction 2765) -> l1_rot5 : {gesamte_autos = berechne_gesamte_autos(counter(1), counter(2), counter(3), counter(4), counter(5), counter(6), counter(7));}
  (junction 1107) -> (junction 1128) : {[autos_auf_spur4, spur4] = autos_auf_spur_generieren(spur4, gesamtZeit + timeCounter, autos_auf_spur4);}
  (junction 3250) -> l1_rot6 : {timer_spuren = countOnwards(timer_spuren,3,[0 0 1 1 1 1 1]);}
  l1_rot3 -> (junction 1728) : after(3,sec)
      | {timeCounter = refresher(timeCounter, 3);}
  (junction 1128) -> (junction 1127) : after(45,sec)
      | {timeCounter = refresher(timeCounter,45);}
  rg1_gelb2 -> (junction 1732) : after(3,sec)
      | {timeCounter = refresher(timeCounter, 3);}
  l1_rot6 -> (junction 3263) : {[anz_autos1, autos_auf_spur1, counter(1), endzeiten1] = generiere_gruenphase(1, 6, autos_auf_spur1, counter(1),  (gesamtZeit + timeCounter - 6), endzeiten1, startzeiten1, auslastung, autos_spur1_flag);}
  l1_rot5 -> (junction 2763) : after(3,sec)
      | {timeCounter = refresher(timeCounter, 3);}
  (junction 1728) -> ampel2_rotgelb1 : {timer_spuren = countOnwards(timer_spuren,3,[1 0 1 1 1 1 1]);}
  rg1_gelb4 -> (junction 2764) : after(3,sec)
      | {timeCounter = refresher(timeCounter, 3);}
  (junction 1127) -> Fuss7_rot : {timer_spuren = countOnwards(timer_spuren,45,[1 0 0 0 1 1 1]);}
  (junction 2763) -> ampel2_rotgelb2 : {timer_spuren = countOnwards(timer_spuren,3,[1 0 1 1 1 1 1]);}
  (junction 3263) -> (junction 3252) : {wartezeiten1 = berechne_wartezeiten(startzeiten1, endzeiten1, alte_counter(1), counter(1), wartezeiten1);}
  (junction 1732) -> (junction 1706) : {[autos_auf_spur2, spur2] = autos_auf_spur_generieren(spur2, gesamtZeit + timeCounter, autos_auf_spur2);}
  ampel2_rotgelb1 -> (junction 1729) : after(1,sec)
      | {timeCounter = refresher(timeCounter, 1);}
  (junction 2764) -> (junction 2768) : {[autos_auf_spur2, spur2] = autos_auf_spur_generieren(spur2, gesamtZeit + timeCounter, autos_auf_spur2);}
  (junction 1124) -> (junction 1121) : {wartezeiten2 = berechne_wartezeiten(startzeiten2, endzeiten2, alte_counter(2), counter(2), wartezeiten2);}
  (junction 3252) -> (junction 3268) : {wartezeit_spur1_ges = gesamt_wartezeit_pro_spur(wartezeiten1, wartezeit_spur1_ges, alte_counter(1), counter(1));}
  Fuss7_rot6 -> (junction 3261) : after(2,sec)
      | {timeCounter = refresher(timeCounter, 2);}
  ampel2_rotgelb2 -> (junction 2766) : after(1,sec)
      | {timeCounter = refresher(timeCounter, 1);}
  (junction 1729) -> ampel2_fuss8_gruen1 : {timer_spuren = countOnwards(timer_spuren,1,[1 0 1 1 1 1 1]);}
  (junction 1706) -> rg1_rot6 : {timer_spuren = countOnwards(timer_spuren,3,[1 0 0 0 1 1 1]);}
  (junction 3268) -> (junction 3262) : {gesamtwartezeit = berechne_gesamtwartezeit(wartezeit_spur1_ges, wartezeit_spur2_ges, wartezeit_spur3_ges, wartezeit_spur4_ges, wartezeit_spur5_ges, wartezeit_spur6_ges, wartezeit_spur7_ges);}
  (junction 2766) -> ampel2_fuss8_gruen2 : {timer_spuren = countOnwards(timer_spuren,1,[1 0 1 1 1 1 1]);}
  (junction 2768) -> rg1_rot13 : {timer_spuren = countOnwards(timer_spuren,3,[1 0 0 0 1 1 1]);}
  (junction 3262) -> l1_rot7 : {gesamte_autos = berechne_gesamte_autos(counter(1), counter(2), counter(3), counter(4), counter(5), counter(6), counter(7));}
  (junction 3261) -> rg1_gelb7 : {timer_spuren = countOnwards(timer_spuren,2,[1 0 0 0 1 1 1]);}
  ampel2_fuss8_gruen1 -> (junction 1733) : {[autos_auf_spur3, spur3] = autos_auf_spur_generieren(spur3, gesamtZeit + timeCounter, autos_auf_spur3);}
  rg1_rot6 -> (junction 1709) : {[anz_autos2, autos_auf_spur2, counter(2), endzeiten2] = generiere_gruenphase(2, 40, autos_auf_spur2, counter(2),  (gesamtZeit + timeCounter - 40), endzeiten2, startzeiten2, auslastung, autos_spur1_flag);}
  Fuss7_rot -> (junction 1114) : after(2,sec)
      | {timeCounter = refresher(timeCounter, 2);}
  rg1_rot13 -> (junction 2771) : {[anz_autos2, autos_auf_spur2, counter(2), endzeiten2] = generiere_gruenphase(2, 25, autos_auf_spur2, counter(2),  (gesamtZeit + timeCounter - 25), endzeiten2, startzeiten2, auslastung, autos_spur1_flag);}
  (junction 1121) -> (junction 1105) : {wartezeit_spur2_ges = gesamt_wartezeit_pro_spur(wartezeiten2, wartezeit_spur2_ges, alte_counter(2), counter(2));}
  ampel2_fuss8_gruen2 -> (junction 2769) : {[autos_auf_spur3, spur3] = autos_auf_spur_generieren(spur3, gesamtZeit + timeCounter, autos_auf_spur3);}
  l1_rot7 -> (junction 3256) : after(3,sec)
      | {timeCounter = refresher(timeCounter, 3);}
  (junction 1114) -> rg1_gelb : {timer_spuren = countOnwards(timer_spuren,2,[1 0 0 0 1 1 1]);}
  rg1_gelb7 -> (junction 3269) : after(2,sec)
      | {timeCounter = refresher(timeCounter, 2);}
  (junction 1733) -> (junction 1707) : {[autos_auf_spur4, spur4] = autos_auf_spur_generieren(spur4, gesamtZeit + timeCounter, autos_auf_spur4);}
  (junction 2769) -> (junction 2767) : {[autos_auf_spur4, spur4] = autos_auf_spur_generieren(spur4, gesamtZeit + timeCounter, autos_auf_spur4);}
  (junction 3256) -> fuss7_rot : {timer_spuren = countOnwards(timer_spuren,3,[1 0 1 1 1 1 1]);}
  (junction 1105) -> (junction 1101) : {gesamtwartezeit = berechne_gesamtwartezeit(wartezeit_spur1_ges, wartezeit_spur2_ges, wartezeit_spur3_ges, wartezeit_spur4_ges, wartezeit_spur5_ges, wartezeit_spur6_ges, wartezeit_spur7_ges)}
  (junction 1707) -> (junction 1713) : after(35,sec)
      | {timeCounter = refresher(timeCounter, 35);}
  (junction 3269) -> (junction 3266) : {[autos_auf_spur2, spur2] = autos_auf_spur_generieren(spur2, gesamtZeit + timeCounter, autos_auf_spur2);}
  rg1_gelb -> (junction 1100) : after(3,sec)
      | {timeCounter = refresher(timeCounter, 3);}
  (junction 2767) -> (junction 2770) : after(10,sec)
      | {timeCounter = refresher(timeCounter, 10);}
  (junction 1713) -> Fuss7_rot3 : {timer_spuren = countOnwards(timer_spuren,35,[1 0 0 0 1 1 1]);}
  (junction 1100) -> (junction 1109) : {[autos_auf_spur2, spur2] = autos_auf_spur_generieren(spur2, gesamtZeit + timeCounter, autos_auf_spur2);}
  (junction 2770) -> Fuss7_rot5 : {timer_spuren = countOnwards(timer_spuren,10,[1 0 0 0 1 1 1]);}
  (junction 3266) -> rg1_rot20 : {timer_spuren = countOnwards(timer_spuren,2,[1 0 0 0 1 1 1]);}
  (junction 1109) -> rg1_rot : {timer_spuren = countOnwards(timer_spuren,3,[1 0 0 0 1 1 1]);}
  (junction 1101) -> rg1_rot5 : {gesamte_autos = berechne_gesamte_autos(counter(1), counter(2), counter(3), counter(4), counter(5), counter(6), counter(7))}
  (junction 1709) -> (junction 1705) : {wartezeiten2 = berechne_wartezeiten(startzeiten2, endzeiten2, alte_counter(2), counter(2), wartezeiten2);}
  (junction 2771) -> (junction 2772) : {wartezeiten2 = berechne_wartezeiten(startzeiten2, endzeiten2, alte_counter(2), counter(2), wartezeiten2);}
  fuss7_rot -> (junction 3253) : after(1,sec)
      | {timeCounter = refresher(timeCounter, 1);}
  rg1_rot20 -> (junction 3270) : {[anz_autos2, autos_auf_spur2, counter(2), endzeiten2] = generiere_gruenphase(2, 9, autos_auf_spur2, counter(2),  (gesamtZeit + timeCounter - 9), endzeiten2, startzeiten2, auslastung, autos_spur1_flag);}
  rg1_rot -> (junction 1125) : {[anz_autos2, autos_auf_spur2, counter(2), endzeiten2] = generiere_gruenphase(2, 65, autos_auf_spur2, counter(2),  (gesamtZeit + timeCounter - 65), endzeiten2, startzeiten2, auslastung, autos_spur1_flag);}
  (junction 3253) -> ampel2_rotgelb3 : {timer_spuren = countOnwards(timer_spuren,1,[1 0 1 1 1 1 1]);}
  Fuss7_rot3 -> (junction 1730) : after(2,sec)
      | {timeCounter = refresher(timeCounter, 2);}
  (junction 1125) -> (junction 1110) : {wartezeiten2 = berechne_wartezeiten(startzeiten2, endzeiten2, alte_counter(2), counter(2), wartezeiten2);}
  (junction 1705) -> (junction 1716) : {wartezeit_spur2_ges = gesamt_wartezeit_pro_spur(wartezeiten2, wartezeit_spur2_ges, alte_counter(2), counter(2));}
  Fuss7_rot5 -> (junction 2779) : after(2,sec)
      | {timeCounter = refresher(timeCounter, 2);}
  rg1_rot5 -> (junction 1122)
  (junction 2772) -> (junction 2781) : {wartezeit_spur2_ges = gesamt_wartezeit_pro_spur(wartezeiten2, wartezeit_spur2_ges, alte_counter(2), counter(2));}
  (junction 1730) -> rg1_gelb3 : {timer_spuren = countOnwards(timer_spuren,2,[1 0 0 0 1 1 1]);}
  ampel2_rotgelb3 -> (junction 3251) : after(1,sec)
      | {timeCounter = refresher(timeCounter, 1);}
  (junction 2779) -> rg1_gelb5 : {timer_spuren = countOnwards(timer_spuren,2,[1 0 0 0 1 1 1]);}
  (junction 1110) -> (junction 1119) : {wartezeit_spur2_ges = gesamt_wartezeit_pro_spur(wartezeiten2, wartezeit_spur2_ges, alte_counter(2), counter(2));}
  (junction 3251) -> ampel2_fuss8_gruen3 : {timer_spuren = countOnwards(timer_spuren,1,[1 0 1 1 1 1 1]);}
  (junction 1716) -> (junction 1735) : {gesamtwartezeit = berechne_gesamtwartezeit(wartezeit_spur1_ges, wartezeit_spur2_ges, wartezeit_spur3_ges, wartezeit_spur4_ges, wartezeit_spur5_ges, wartezeit_spur6_ges, wartezeit_spur7_ges)}
  (junction 2781) -> (junction 2775) : {gesamtwartezeit = berechne_gesamtwartezeit(wartezeit_spur1_ges, wartezeit_spur2_ges, wartezeit_spur3_ges, wartezeit_spur4_ges, wartezeit_spur5_ges, wartezeit_spur6_ges, wartezeit_spur7_ges)}
  rg1_gelb3 -> (junction 1717) : after(3,sec)
      | {timeCounter = refresher(timeCounter, 3);}
  (junction 3270) -> (junction 3255) : {wartezeiten2 = berechne_wartezeiten(startzeiten2, endzeiten2, alte_counter(2), counter(2), wartezeiten2);}
  rg1_gelb5 -> (junction 2780) : after(3,sec)
      | {timeCounter = refresher(timeCounter, 3);}
  (junction 1717) -> (junction 1734) : {[autos_auf_spur2, spur2] = autos_auf_spur_generieren(spur2, gesamtZeit + timeCounter, autos_auf_spur2);}
  (junction 1119) -> (junction 1104) : {gesamtwartezeit = berechne_gesamtwartezeit(wartezeit_spur1_ges, wartezeit_spur2_ges, wartezeit_spur3_ges, wartezeit_spur4_ges, wartezeit_spur5_ges, wartezeit_spur6_ges, wartezeit_spur7_ges)}
  (junction 2780) -> (junction 2776) : {[autos_auf_spur2, spur2] = autos_auf_spur_generieren(spur2, gesamtZeit + timeCounter, autos_auf_spur2);}
  (junction 1734) -> rg1_rot7 : {timer_spuren = countOnwards(timer_spuren,3,[1 0 0 0 1 1 1]);}
  (junction 1735) -> rg1_rot11 : {gesamte_autos = berechne_gesamte_autos(counter(1), counter(2), counter(3), counter(4), counter(5), counter(6), counter(7))}
  ampel2_fuss8_gruen3 -> (junction 3254) : {[autos_auf_spur3, spur3] = autos_auf_spur_generieren(spur3, gesamtZeit + timeCounter, autos_auf_spur3);}
  (junction 2775) -> fuss8_rot7 : {gesamte_autos = berechne_gesamte_autos(counter(1), counter(2), counter(3), counter(4), counter(5), counter(6), counter(7))}
  (junction 2776) -> rg1_rot14 : {timer_spuren = countOnwards(timer_spuren,3,[1 0 0 0 1 1 1]);}
  (junction 1104) -> rg1_rot4 : {gesamte_autos = berechne_gesamte_autos(counter(1), counter(2), counter(3), counter(4), counter(5), counter(6), counter(7))}
  (junction 3254) -> rg1_gelb6 : {[autos_auf_spur4, spur4] = autos_auf_spur_generieren(spur4, gesamtZeit + timeCounter, autos_auf_spur4);}
  rg1_rot7 -> (junction 1710) : {[anz_autos2, autos_auf_spur2, counter(2), endzeiten2] = generiere_gruenphase(2, 55, autos_auf_spur2, counter(2),  (gesamtZeit + timeCounter - 55), endzeiten2, startzeiten2, auslastung, autos_spur1_flag);}
  (junction 3255) -> (junction 3257) : {wartezeit_spur2_ges = gesamt_wartezeit_pro_spur(wartezeiten2, wartezeit_spur2_ges, alte_counter(2), counter(2));}
  rg1_rot14 -> (junction 2773) : {[anz_autos2, autos_auf_spur2, counter(2), endzeiten2] = generiere_gruenphase(2, 30, autos_auf_spur2, counter(2),  (gesamtZeit + timeCounter - 30), endzeiten2, startzeiten2, auslastung, autos_spur1_flag);}
  rg1_rot4 -> (junction 1113)
  (junction 1710) -> (junction 1714) : {wartezeiten2 = berechne_wartezeiten(startzeiten2, endzeiten2, alte_counter(2), counter(2), wartezeiten2);}
  rg1_gelb6 -> (junction 3271) : after(3,sec)
      | {timeCounter = refresher(timeCounter, 3);}
  (junction 2773) -> (junction 2777) : {wartezeiten2 = berechne_wartezeiten(startzeiten2, endzeiten2, alte_counter(2), counter(2), wartezeiten2);}
  rg1_rot11 -> (junction 1762)
  (junction 3257) -> (junction 3273) : {gesamtwartezeit = berechne_gesamtwartezeit(wartezeit_spur1_ges, wartezeit_spur2_ges, wartezeit_spur3_ges, wartezeit_spur4_ges, wartezeit_spur5_ges, wartezeit_spur6_ges, wartezeit_spur7_ges)}
  fuss8_rot7 -> (junction 2784)
  (junction 3271) -> (junction 3272) : {[autos_auf_spur2, spur2] = autos_auf_spur_generieren(spur2, gesamtZeit + timeCounter, autos_auf_spur2);}
  (junction 1714) -> (junction 1718) : {wartezeit_spur2_ges = gesamt_wartezeit_pro_spur(wartezeiten2, wartezeit_spur2_ges, alte_counter(2), counter(2));}
  (junction 3272) -> rg1_rot17 : {timer_spuren = countOnwards(timer_spuren,3,[1 0 0 0 1 1 1]);}
  (junction 2777) -> (junction 2778) : {wartezeit_spur2_ges = gesamt_wartezeit_pro_spur(wartezeiten2, wartezeit_spur2_ges, alte_counter(2), counter(2));}
  (junction 3273) -> fuss8_rot11 : {gesamte_autos = berechne_gesamte_autos(counter(1), counter(2), counter(3), counter(4), counter(5), counter(6), counter(7))}
  rg1_rot17 -> (junction 3104) : {[anz_autos2, autos_auf_spur2, counter(2), endzeiten2] = generiere_gruenphase(2, 13, autos_auf_spur2, counter(2),  (gesamtZeit + timeCounter - 13 ), endzeiten2, startzeiten2, auslastung, autos_spur1_flag);}
  (junction 1113) -> (junction 1111)
  (junction 1122) -> (junction 1113)
  (junction 1718) -> (junction 1757) : {gesamtwartezeit = berechne_gesamtwartezeit(wartezeit_spur1_ges, wartezeit_spur2_ges, wartezeit_spur3_ges, wartezeit_spur4_ges, wartezeit_spur5_ges, wartezeit_spur6_ges, wartezeit_spur7_ges)}
  (junction 1111) -> (junction 1112)
  (junction 2778) -> (junction 2774) : {gesamtwartezeit = berechne_gesamtwartezeit(wartezeit_spur1_ges, wartezeit_spur2_ges, wartezeit_spur3_ges, wartezeit_spur4_ges, wartezeit_spur5_ges, wartezeit_spur6_ges, wartezeit_spur7_ges)}
  (junction 3104) -> (junction 3101) : {wartezeiten2 = berechne_wartezeiten(startzeiten2, endzeiten2, alte_counter(2), counter(2), wartezeiten2);}
  (junction 1757) -> rg1_rot9 : {gesamte_autos = berechne_gesamte_autos(counter(1), counter(2), counter(3), counter(4), counter(5), counter(6), counter(7))}
  (junction 2774) -> rg1_rot12 : {gesamte_autos = berechne_gesamte_autos(counter(1), counter(2), counter(3), counter(4), counter(5), counter(6), counter(7))}
  (junction 3101) -> (junction 3094) : {wartezeit_spur2_ges = gesamt_wartezeit_pro_spur(wartezeiten2, wartezeit_spur2_ges, alte_counter(2), counter(2));}
  fuss8_rot11 -> (junction 3102) : after(2,sec)
      | {timeCounter = refresher(timeCounter, 1);}
  rg1_rot9 -> (junction 1764)
  rg1_rot12 -> (junction 2799)
  (junction 3102) -> (junction 3103) : {timer_spuren = countOnwards(timer_spuren,2,[1 1 0 0 1 1 1]);}
  (junction 3094) -> (junction 3096) : {gesamtwartezeit = berechne_gesamtwartezeit(wartezeit_spur1_ges, wartezeit_spur2_ges, wartezeit_spur3_ges, wartezeit_spur4_ges, wartezeit_spur5_ges, wartezeit_spur6_ges, wartezeit_spur7_ges)}
  (junction 3096) -> rg1_rot21 : {gesamte_autos = berechne_gesamte_autos(counter(1), counter(2), counter(3), counter(4), counter(5), counter(6), counter(7))}
  (junction 1764) -> (junction 1741)
  (junction 1762) -> (junction 1764)
  (junction 1741) -> (junction 1751)
  (junction 2784) -> fuss8_rot8 [order 1] : [autos_auf_spur3 <= 2]
  (junction 2784) -> (junction 2806) [order 2]
  (junction 2786) -> (junction 2659)
  (junction 2799) -> rg1_rot16 [order 1] : [autos_auf_spur3 <= 2]
  rg1_rot21 -> (junction 3095)
  (junction 2799) -> (junction 2801) [order 2]
  fuss8_rot8 -> (junction 2787) : %after(2,sec)
      | %{timeCounter = refresher(timeCounter, 2);}
  rg1_rot16 -> (junction 2785) : %after(10,sec)
      | %{timeCounter = refresher(timeCounter, 10);}
  (junction 2806) -> fuss8_rot9 [order 1] : [autos_auf_spur3 > 2]
  (junction 2806) -> (junction 2844) [order 2]
  (junction 2801) -> rg1_rot15 [order 1] : [autos_auf_spur3 > 2]
  (junction 2801) -> (junction 2677) [order 2]
  rg1_rot15 -> (junction 2797) : after(15,sec)
      | {timeCounter = refresher(timeCounter, 15);}
  fuss8_rot9 -> (junction 2800) : after(10,sec)
      | {timeCounter = refresher(timeCounter, 10);}
  (junction 2785) -> fuss8_rot5 : %{timer_spuren = countOnwards(timer_spuren,10,[1 1 0 0 1 1 1]);}
  (junction 2797) -> fuss8_rot4 : {timer_spuren = countOnwards(timer_spuren,15,[1 1 0 0 1 1 1]);}
  fuss8_rot5 -> (junction 2782) : after(2,sec)
      | {timeCounter = refresher(timeCounter, 2);}
  (junction 3095) -> rg1_rot19 [order 1] : [autos_auf_spur3 <= 2]
  (junction 3095) -> (junction 3097) [order 2]
  (junction 3103) -> ampel2_gelb8 [order 1] : [autos_auf_spur3 <= 2]
  (junction 2787) -> ampel2_gelb6 : %{timer_spuren = countOnwards(timer_spuren,2,[1 1 0 0 1 1 1]);}
  (junction 3103) -> (junction 3098) [order 2]
  fuss8_rot4 -> (junction 2802) : after(2,sec)
      | {timeCounter = refresher(timeCounter, 2);}
  rg1_rot19 -> (junction 3099) : after(3,sec)
      | {timeCounter = refresher(timeCounter, 3);}
  ampel2_gelb8 -> (junction 3118) : after(3,sec)
      | {timeCounter = refresher(timeCounter, 3);}
  (junction 2800) -> ampel2_gelb7 : {timer_spuren = countOnwards(timer_spuren,10,[1 1 0 0 1 1 1]);}
  (junction 2782) -> ampel2_gelb5 : {timer_spuren = countOnwards(timer_spuren,2,[1 1 0 0 1 1 1]);}
  (junction 1112) -> rg1_rot3 [order 1] : [autos_auf_spur3 <= 2]
  (junction 1112) -> (junction 1115) [order 2]
  (junction 2802) -> ampel2_gelb4 : {timer_spuren = countOnwards(timer_spuren,2,[1 1 0 0 1 1 1]);}
  (junction 3097) -> rg1_rot18 [order 1] : [autos_auf_spur3 > 2]
  (junction 3097) -> (junction 3176) [order 2]
  rg1_rot3 -> (junction 1120) : after(7,sec)
      | {timeCounter = refresher(timeCounter, 7);}
  (junction 3098) -> ampel2_gelb11 [order 1] : [autos_auf_spur3 > 2]
  rg1_rot18 -> (junction 3100) : after(3,sec)
      | {timeCounter = refresher(timeCounter, 3);}
  (junction 3098) -> (junction 3184) [order 2]
  ampel2_gelb6 -> (junction 2788) : %after(3,sec)
      | %{timeCounter = refresher(timeCounter, 3);}
  (junction 1115) -> rg1_rot2 [order 1] : [autos_auf_spur3 > 2]
  ampel2_gelb11 -> (junction 3117) : after(3,sec)
      | {timeCounter = refresher(timeCounter, 3);}
  (junction 1115) -> (junction 1138) [order 2]
  (junction 3099) -> fuss8_rot10 : {timer_spuren = countOnwards(timer_spuren,3,[1 1 0 0 1 1 1]);}
  ampel2_gelb7 -> (junction 2793) : after(3,sec)
      | {timeCounter = refresher(timeCounter, 3);}
  ampel2_gelb5 -> (junction 2789) : after(3,sec)
      | {timeCounter = refresher(timeCounter, 3);}
  rg1_rot2 -> (junction 1116) : after(20,sec)
      | {timeCounter = refresher(timeCounter, 20);}
  ampel2_gelb4 -> (junction 2791) : after(3,sec)
      | {timeCounter = refresher(timeCounter, 3);}
  (junction 2793) -> (junction 2803) : {timer_spuren = countOnwards(timer_spuren,3,[1 1 0 0 1 1 1]);}
  (junction 2788) -> (junction 2804) : %{timer_spuren = countOnwards(timer_spuren,3,[1 1 0 0 1 1 1]);}
  (junction 1120) -> fuss8_rot1 : {timer_spuren = countOnwards(timer_spuren,7,[1 1 0 0 1 1 1]);}
  (junction 2791) -> (junction 2798) : {timer_spuren = countOnwards(timer_spuren,3,[1 1 0 0 1 1 1]);}
  (junction 2789) -> (junction 2795) : {timer_spuren = countOnwards(timer_spuren,3,[1 1 0 0 1 1 1]);}
  (junction 3100) -> fuss8_rot12 : {timer_spuren = countOnwards(timer_spuren,3,[1 1 0 0 1 1 1]);}
  (junction 2803) -> (junction 2807) : {[autos_auf_spur3, spur3] = autos_auf_spur_generieren(spur3, gesamtZeit + timeCounter, autos_auf_spur3);}
  (junction 2804) -> (junction 2809) : {[autos_auf_spur3, spur3] = autos_auf_spur_generieren(spur3, gesamtZeit + timeCounter, autos_auf_spur3);}
  (junction 1116) -> fuss8_rot : {timer_spuren = countOnwards(timer_spuren,20,[1 1 0 0 1 1 1]);}
  (junction 2798) -> (junction 2810) : {[autos_auf_spur3, spur3] = autos_auf_spur_generieren(spur3, gesamtZeit + timeCounter, autos_auf_spur3);}
  (junction 2795) -> (junction 2790) : {[autos_auf_spur3, spur3] = autos_auf_spur_generieren(spur3, gesamtZeit + timeCounter, autos_auf_spur3);}
  fuss8_rot10 -> (junction 3127) : after(2,sec)
      | {timeCounter = refresher(timeCounter, 2);}
  (junction 2807) -> ampel2_rot12 : {[autos_auf_spur4, spur4] = autos_auf_spur_generieren(spur4, gesamtZeit + timeCounter, autos_auf_spur4);}
  fuss8_rot12 -> (junction 3107) : after(2,sec)
      | {timeCounter = refresher(timeCounter, 2);}
  fuss8_rot1 -> (junction 1106) : after(2,sec)
      | {timeCounter = refresher(timeCounter, 2);}
  (junction 2810) -> ampel2_rot11 : {[autos_auf_spur4, spur4] = autos_auf_spur_generieren(spur4, gesamtZeit + timeCounter, autos_auf_spur4);}
  (junction 3127) -> ampel2_gelb9 : {timer_spuren = countOnwards(timer_spuren,2,[1 1 0 0 1 1 1]);}
  (junction 2809) -> ampel2_rot13 : {[autos_auf_spur4, spur4] = autos_auf_spur_generieren(spur4, gesamtZeit + timeCounter, autos_auf_spur4);}
  (junction 3107) -> ampel2_gelb10 : {timer_spuren = countOnwards(timer_spuren,2,[1 1 0 0 1 1 1]);}
  fuss8_rot -> (junction 1108) : after(2,sec)
      | {timeCounter = refresher(timeCounter, 2);}
  (junction 2790) -> ampel2_rot9 : {[autos_auf_spur4, spur4] = autos_auf_spur_generieren(spur4, gesamtZeit + timeCounter, autos_auf_spur4);}
  (junction 1106) -> ampel2_gelb1 : {timer_spuren = countOnwards(timer_spuren,2,[1 1 0 0 1 1 1]);}
  (junction 1108) -> ampel2_gelb : {timer_spuren = countOnwards(timer_spuren,2,[1 1 0 0 1 1 1]);}
  ampel2_rot12 -> (junction 2783) : {[anz_autos3, autos_auf_spur3, counter(3), endzeiten3] = generiere_gruenphase(3, 40, autos_auf_spur3, counter(3),  (gesamtZeit + timeCounter - 40), endzeiten3, startzeiten3, auslastung, autos_spur1_flag)}
  ampel2_gelb9 -> (junction 3112) : after(3,sec)
      | {timeCounter = refresher(timeCounter, 3);}
  ampel2_rot11 -> (junction 2805) : {[anz_autos3, autos_auf_spur3, counter(3), endzeiten3] = generiere_gruenphase(3, 35, autos_auf_spur3, counter(3),  (gesamtZeit + timeCounter -  35), endzeiten3, startzeiten3, auslastung, autos_spur1_flag)}
  ampel2_gelb10 -> (junction 3124) : after(3,sec)
      | {timeCounter = refresher(timeCounter, 3);}
  (junction 1751) -> rg1_rot8 [order 1] : [autos_auf_spur3 <= 2]
  (junction 1751) -> (junction 1742) [order 2]
  ampel2_gelb1 -> (junction 1130) : after(3,sec)
      | {timeCounter = refresher(timeCounter, 3);}
  (junction 3124) -> (junction 3125) : {timer_spuren = countOnwards(timer_spuren,3,[1 1 0 0 1 1 1]);}
  (junction 3112) -> (junction 3113) : {timer_spuren = countOnwards(timer_spuren,3,[1 1 0 0 1 1 1]);}
  rg1_rot8 -> (junction 1744) : after(7,sec)
      | {timeCounter = refresher(timeCounter, 7);}
  ampel2_gelb -> (junction 1129) : after(3,sec)
      | {timeCounter = refresher(timeCounter, 3);}
  (junction 1742) -> rg1_rot10 [order 1] : [autos_auf_spur3 > 2]
  (junction 3117) -> (junction 3126) : {timer_spuren = countOnwards(timer_spuren,3,[1 1 0 0 1 1 1]);}
  (junction 3118) -> (junction 3114) : {timer_spuren = countOnwards(timer_spuren,3,[1 1 0 0 1 1 1]);}
  (junction 1742) -> (junction 1768) [order 2]
  (junction 1129) -> (junction 1126) : {timer_spuren = countOnwards(timer_spuren,3,[1 1 0 0 1 1 1]);}
  (junction 1130) -> (junction 1123) : {timer_spuren = countOnwards(timer_spuren,3,[1 1 0 0 1 1 1]);}
  rg1_rot10 -> (junction 1739) : after(20,sec)
      | {timeCounter = refresher(timeCounter, 20);}
  (junction 2783) -> (junction 2792) : {wartezeiten3 = berechne_wartezeiten(startzeiten3, endzeiten3, alte_counter(3), counter(3), wartezeiten3);}
  (junction 3125) -> (junction 3119) : {[autos_auf_spur3, spur3] = autos_auf_spur_generieren(spur3, gesamtZeit + timeCounter, autos_auf_spur3);}
  (junction 3113) -> (junction 3115) : {[autos_auf_spur3, spur3] = autos_auf_spur_generieren(spur3, gesamtZeit + timeCounter, autos_auf_spur3);}
  (junction 2805) -> (junction 2796) : {wartezeiten3 = berechne_wartezeiten(startzeiten3, endzeiten3, alte_counter(3), counter(3), wartezeiten3);}
  (junction 1744) -> fuss8_rot3 : {timer_spuren = countOnwards(timer_spuren,7,[1 1 0 0 1 1 1]);}
  (junction 3126) -> (junction 3106) : {[autos_auf_spur3, spur3] = autos_auf_spur_generieren(spur3, gesamtZeit + timeCounter, autos_auf_spur3);}
  (junction 3114) -> (junction 3111) : {[autos_auf_spur3, spur3] = autos_auf_spur_generieren(spur3, gesamtZeit + timeCounter, autos_auf_spur3);}
  (junction 1126) -> (junction 1117) : {[autos_auf_spur3, spur3] = autos_auf_spur_generieren(spur3, gesamtZeit + timeCounter, autos_auf_spur3);}
  (junction 1123) -> (junction 1118) : {[autos_auf_spur3, spur3] = autos_auf_spur_generieren(spur3, gesamtZeit + timeCounter, autos_auf_spur3);}
  (junction 3119) -> ampel2_rot19 : {[autos_auf_spur4, spur4] = autos_auf_spur_generieren(spur4, gesamtZeit + timeCounter, autos_auf_spur4);}
  (junction 3120) -> (junction 3108)
  (junction 2792) -> (junction 2794) : {wartezeit_spur3_ges = gesamt_wartezeit_pro_spur(wartezeiten3, wartezeit_spur3_ges, alte_counter(3), counter(3));}
  (junction 1739) -> fuss8_rot2 : {timer_spuren = countOnwards(timer_spuren,20,[1 1 0 0 1 1 1]);}
  (junction 3106) -> ampel2_rot17 : {[autos_auf_spur4, spur4] = autos_auf_spur_generieren(spur4, gesamtZeit + timeCounter, autos_auf_spur4);}
  (junction 3115) -> ampel2_rot21 : {[autos_auf_spur4, spur4] = autos_auf_spur_generieren(spur4, gesamtZeit + timeCounter, autos_auf_spur4);}
  (junction 2796) -> (junction 2820) : {wartezeit_spur3_ges = gesamt_wartezeit_pro_spur(wartezeiten3, wartezeit_spur3_ges, alte_counter(3), counter(3));}
  (junction 1117) -> ampel2_rot : {[autos_auf_spur4, spur4] = autos_auf_spur_generieren(spur4, gesamtZeit + timeCounter, autos_auf_spur4);}
  ampel2_rot13 -> (junction 2808) : {[anz_autos3, autos_auf_spur3, counter(3), endzeiten3] = generiere_gruenphase(3, 25, autos_auf_spur3, counter(3),  (gesamtZeit + timeCounter - 25), endzeiten3, startzeiten3, auslastung, autos_spur1_flag)}
  (junction 3111) -> ampel2_rot20 : {[autos_auf_spur4, spur4] = autos_auf_spur_generieren(spur4, gesamtZeit + timeCounter, autos_auf_spur4);}
  ampel2_rot9 -> (junction 2818) : {[anz_autos3, autos_auf_spur3, counter(3), endzeiten3] = generiere_gruenphase(3, 20, autos_auf_spur3, counter(3),  (gesamtZeit + timeCounter - 20), endzeiten3, startzeiten3, auslastung, autos_spur1_flag)}
  (junction 1118) -> ampel2_rot1 : {[autos_auf_spur4, spur4] = autos_auf_spur_generieren(spur4, gesamtZeit + timeCounter, autos_auf_spur4);}
  ampel2_rot19 -> (junction 3109) : {[anz_autos3, autos_auf_spur3, counter(3), endzeiten3] = generiere_gruenphase(3, 11, autos_auf_spur3, counter(3),  (gesamtZeit + timeCounter - 11), endzeiten3, startzeiten3, auslastung, autos_spur1_flag);}
  fuss8_rot3 -> (junction 1738) : after(2,sec)
      | {timeCounter = refresher(timeCounter, 2);}
  (junction 2794) -> (junction 2813) : {gesamtwartezeit = berechne_gesamtwartezeit(wartezeit_spur1_ges, wartezeit_spur2_ges, wartezeit_spur3_ges, wartezeit_spur4_ges, wartezeit_spur5_ges, wartezeit_spur6_ges, wartezeit_spur7_ges);}
  (junction 2808) -> (junction 2819) : {wartezeiten3 = berechne_wartezeiten(startzeiten3, endzeiten3, alte_counter(3), counter(3), wartezeiten3);}
  ampel2_rot17 -> (junction 3123) : {[anz_autos3, autos_auf_spur3, counter(3), endzeiten3] = generiere_gruenphase(3, 14, autos_auf_spur3, counter(3),  (gesamtZeit + timeCounter - 14), endzeiten3, startzeiten3, auslastung, autos_spur1_flag);}
  fuss8_rot2 -> (junction 1748) : after(2,sec)
      | {timeCounter = refresher(timeCounter, 2);}
  (junction 2820) -> (junction 2812) : {gesamtwartezeit = berechne_gesamtwartezeit(wartezeit_spur1_ges, wartezeit_spur2_ges, wartezeit_spur3_ges, wartezeit_spur4_ges, wartezeit_spur5_ges, wartezeit_spur6_ges, wartezeit_spur7_ges);}
  (junction 3108) -> (junction 3121)
  ampel2_rot -> (junction 1102) : {[anz_autos3, autos_auf_spur3, counter(3), endzeiten3] = generiere_gruenphase(3, 75, autos_auf_spur3, counter(3),  (gesamtZeit + timeCounter - 75), endzeiten3, startzeiten3, auslastung, autos_spur1_flag);}
  (junction 2818) -> (junction 2811) : {wartezeiten3 = berechne_wartezeiten(startzeiten3, endzeiten3, alte_counter(3), counter(3), wartezeiten3);}
  (junction 1738) -> ampel2_gelb3 : {timer_spuren = countOnwards(timer_spuren,2,[1 1 0 0 1 1 1]);}
  (junction 1748) -> ampel2_gelb2 : {timer_spuren = countOnwards(timer_spuren,2,[1 1 0 0 1 1 1]);}
  (junction 2813) -> (junction 2814) : {gesamte_autos = berechne_gesamte_autos(counter(1), counter(2), counter(3), counter(4), counter(5), counter(6), counter(7));}
  (junction 3121) -> (junction 3186)
  (junction 2812) -> (junction 2817) : {gesamte_autos = berechne_gesamte_autos(counter(1), counter(2), counter(3), counter(4), counter(5), counter(6), counter(7));}
  (junction 2819) -> (junction 2815) : {wartezeit_spur3_ges = gesamt_wartezeit_pro_spur(wartezeiten3, wartezeit_spur3_ges, alte_counter(3), counter(3));}
  (junction 3109) -> (junction 3122) : {wartezeiten3 = berechne_wartezeiten(startzeiten3, endzeiten3, alte_counter(3), counter(3), wartezeiten3);}
  (junction 2811) -> (junction 2816) : {wartezeit_spur3_ges = gesamt_wartezeit_pro_spur(wartezeiten3, wartezeit_spur3_ges, alte_counter(3), counter(3));}
  ampel2_gelb3 -> (junction 1765) : after(3,sec)
      | {timeCounter = refresher(timeCounter, 3);}
  ampel2_gelb2 -> (junction 1746) : after(3,sec)
      | {timeCounter = refresher(timeCounter, 3);}
  (junction 3123) -> (junction 3110) : {wartezeiten3 = berechne_wartezeiten(startzeiten3, endzeiten3, alte_counter(3), counter(3), wartezeiten3);}
  (junction 2814) -> (junction 2823) : {[anz_autos4, autos_auf_spur4, counter(4), endzeiten4] = generiere_gruenphase(4, 40, autos_auf_spur4, counter(4),  (gesamtZeit + timeCounter - 40), endzeiten4, startzeiten4, autos_spur1_flag)}
  (junction 1102) -> (junction 1131) : {wartezeiten3 = berechne_wartezeiten(startzeiten3, endzeiten3, alte_counter(3), counter(3), wartezeiten3);}
  (junction 2817) -> (junction 2824) : {[anz_autos4, autos_auf_spur4, counter(4), endzeiten4] = generiere_gruenphase(4, 35, autos_auf_spur4, counter(4),  (gesamtZeit + timeCounter - 35), endzeiten4, startzeiten4, autos_spur1_flag)}
  (junction 1746) -> (junction 1760) : {timer_spuren = countOnwards(timer_spuren,3,[1 1 0 0 1 1 1]);}
  (junction 1765) -> (junction 1758) : {timer_spuren = countOnwards(timer_spuren,3,[1 1 0 0 1 1 1]);}
  (junction 2815) -> (junction 2821) : {gesamtwartezeit = berechne_gesamtwartezeit(wartezeit_spur1_ges, wartezeit_spur2_ges, wartezeit_spur3_ges, wartezeit_spur4_ges, wartezeit_spur5_ges, wartezeit_spur6_ges, wartezeit_spur7_ges);}
  (junction 3122) -> (junction 3116) : {wartezeit_spur3_ges = gesamt_wartezeit_pro_spur(wartezeiten3, wartezeit_spur3_ges, alte_counter(3), counter(3));}
  (junction 2816) -> (junction 2825) : {gesamtwartezeit = berechne_gesamtwartezeit(wartezeit_spur1_ges, wartezeit_spur2_ges, wartezeit_spur3_ges, wartezeit_spur4_ges, wartezeit_spur5_ges, wartezeit_spur6_ges, wartezeit_spur7_ges)}
  (junction 2823) -> (junction 2822) : {wartezeiten4 = berechne_wartezeiten(startzeiten4, endzeiten4, alte_counter(4), counter(4), wartezeiten4);}
  (junction 3110) -> (junction 3147) : {wartezeit_spur3_ges = gesamt_wartezeit_pro_spur(wartezeiten3, wartezeit_spur3_ges, alte_counter(3), counter(3));}
  ampel2_rot21 -> (junction 3105) : {[anz_autos3, autos_auf_spur3, counter(3), endzeiten3] = generiere_gruenphase(3, 11, autos_auf_spur3, counter(3),  (gesamtZeit + timeCounter - 11), endzeiten3, startzeiten3, auslastung, autos_spur1_flag);}
  (junction 1131) -> (junction 1103) : {wartezeit_spur3_ges = gesamt_wartezeit_pro_spur(wartezeiten3, wartezeit_spur3_ges, alte_counter(3), counter(3));}
  (junction 2824) -> (junction 2828) : {wartezeiten4 = berechne_wartezeiten(startzeiten4, endzeiten4, alte_counter(4), counter(4), wartezeiten4);}
  (junction 1760) -> (junction 1753) : {[autos_auf_spur3, spur3] = autos_auf_spur_generieren(spur3, gesamtZeit + timeCounter, autos_auf_spur3);}
  (junction 1758) -> (junction 1743) : {[autos_auf_spur3, spur3] = autos_auf_spur_generieren(spur3, gesamtZeit + timeCounter, autos_auf_spur3);}
  ampel2_rot20 -> (junction 3153) : {[anz_autos3, autos_auf_spur3, counter(3), endzeiten3] = generiere_gruenphase(3, 14, autos_auf_spur3, counter(3),  (gesamtZeit + timeCounter - 14), endzeiten3, startzeiten3, auslastung, autos_spur1_flag);}
  (junction 2821) -> (junction 2826) : {gesamte_autos = berechne_gesamte_autos(counter(1), counter(2), counter(3), counter(4), counter(5), counter(6), counter(7));}
  ampel2_rot1 -> (junction 1158) : {[anz_autos3, autos_auf_spur3, counter(3), endzeiten3] = generiere_gruenphase(3, 62, autos_auf_spur3, counter(3),  (gesamtZeit + timeCounter - 62), endzeiten3, startzeiten3, auslastung, autos_spur1_flag);}
  (junction 2825) -> (junction 2827) : {gesamte_autos = berechne_gesamte_autos(counter(1), counter(2), counter(3), counter(4), counter(5), counter(6), counter(7));}
  (junction 3116) -> (junction 3136) : {gesamtwartezeit = berechne_gesamtwartezeit(wartezeit_spur1_ges, wartezeit_spur2_ges, wartezeit_spur3_ges, wartezeit_spur4_ges, wartezeit_spur5_ges, wartezeit_spur6_ges, wartezeit_spur7_ges);}
  (junction 3105) -> (junction 3139) : {wartezeiten3 = berechne_wartezeiten(startzeiten3, endzeiten3, alte_counter(3), counter(3), wartezeiten3);}
  (junction 2822) -> (junction 2831) : {wartezeit_spur4_ges = gesamt_wartezeit_pro_spur(wartezeiten4, wartezeit_spur4_ges, alte_counter(4), counter(4));}
  (junction 2826) -> (junction 2834) : {[anz_autos4, autos_auf_spur4, counter(4), endzeiten4] = generiere_gruenphase(4, 25, autos_auf_spur4, counter(4),  (gesamtZeit + timeCounter - 25), endzeiten4, startzeiten4, auslastung, autos_spur1_flag)}
  (junction 1753) -> ampel2_rot5 : {[autos_auf_spur4, spur4] = autos_auf_spur_generieren(spur4, gesamtZeit + timeCounter, autos_auf_spur4);}
  (junction 3147) -> (junction 3140) : {gesamtwartezeit = berechne_gesamtwartezeit(wartezeit_spur1_ges, wartezeit_spur2_ges, wartezeit_spur3_ges, wartezeit_spur4_ges, wartezeit_spur5_ges, wartezeit_spur6_ges, wartezeit_spur7_ges);}
  (junction 2828) -> (junction 2829) : {wartezeit_spur4_ges = gesamt_wartezeit_pro_spur(wartezeiten4, wartezeit_spur4_ges, alte_counter(4), counter(4));}
  (junction 2827) -> (junction 2830) : {[anz_autos4, autos_auf_spur4, counter(4), endzeiten4] = generiere_gruenphase(4, 20, autos_auf_spur4, counter(4),  (gesamtZeit + timeCounter - 20), endzeiten4, startzeiten4, auslastung, autos_spur1_flag);}
  (junction 1103) -> (junction 1143) : {gesamtwartezeit = berechne_gesamtwartezeit(wartezeit_spur1_ges, wartezeit_spur2_ges, wartezeit_spur3_ges, wartezeit_spur4_ges, wartezeit_spur5_ges, wartezeit_spur6_ges, wartezeit_spur7_ges);}
  (junction 3153) -> (junction 3156) : {wartezeiten3 = berechne_wartezeiten(startzeiten3, endzeiten3, alte_counter(3), counter(3), wartezeiten3);}
  (junction 1743) -> ampel2_rot6 : {[autos_auf_spur4, spur4] = autos_auf_spur_generieren(spur4, gesamtZeit + timeCounter, autos_auf_spur4);}
  (junction 1158) -> (junction 1153) : {wartezeiten3 = berechne_wartezeiten(startzeiten3, endzeiten3, alte_counter(3), counter(3), wartezeiten3);}
  (junction 2834) -> (junction 2832) : {wartezeiten4 = berechne_wartezeiten(startzeiten4, endzeiten4, alte_counter(4), counter(4), wartezeiten4);}
  (junction 3136) -> (junction 3152) : {gesamte_autos = berechne_gesamte_autos(counter(1), counter(2), counter(3), counter(4), counter(5), counter(6), counter(7));}
  (junction 2830) -> (junction 2833) : {wartezeiten4 = berechne_wartezeiten(startzeiten4, endzeiten4, alte_counter(4), counter(4), wartezeiten4);}
  (junction 3139) -> (junction 3142) : {wartezeit_spur3_ges = gesamt_wartezeit_pro_spur(wartezeiten3, wartezeit_spur3_ges, alte_counter(3), counter(3));}
  (junction 3140) -> (junction 3128) : {gesamte_autos = berechne_gesamte_autos(counter(1), counter(2), counter(3), counter(4), counter(5), counter(6), counter(7));}
  (junction 2831) -> (junction 2837) : {gesamtwartezeit = berechne_gesamtwartezeit(wartezeit_spur1_ges, wartezeit_spur2_ges, wartezeit_spur3_ges, wartezeit_spur4_ges, wartezeit_spur5_ges, wartezeit_spur6_ges, wartezeit_spur7_ges);}
  ampel2_rot5 -> (junction 1747) : {[anz_autos3, autos_auf_spur3, counter(3), endzeiten3] = generiere_gruenphase(3, 65, autos_auf_spur3, counter(3),  (gesamtZeit + timeCounter - 65), endzeiten3, startzeiten3, auslastung, autos_spur1_flag);}
  (junction 1143) -> (junction 1137) : {gesamte_autos = berechne_gesamte_autos(counter(1), counter(2), counter(3), counter(4), counter(5), counter(6), counter(7));}
  (junction 3156) -> (junction 3129) : {wartezeit_spur3_ges = gesamt_wartezeit_pro_spur(wartezeiten3, wartezeit_spur3_ges, alte_counter(3), counter(3));}
  (junction 2829) -> (junction 2838) : {gesamtwartezeit = berechne_gesamtwartezeit(wartezeit_spur1_ges, wartezeit_spur2_ges, wartezeit_spur3_ges, wartezeit_spur4_ges, wartezeit_spur5_ges, wartezeit_spur6_ges, wartezeit_spur7_ges);}
  (junction 2832) -> (junction 2841) : {wartezeit_spur4_ges = gesamt_wartezeit_pro_spur(wartezeiten4, wartezeit_spur4_ges, alte_counter(4), counter(4));}
  (junction 1153) -> (junction 1144) : {wartezeit_spur3_ges = gesamt_wartezeit_pro_spur(wartezeiten3, wartezeit_spur3_ges, alte_counter(3), counter(3));}
  (junction 3152) -> (junction 3131) : {[anz_autos4, autos_auf_spur4, counter(4), endzeiten4] = generiere_gruenphase(4, 55, autos_auf_spur4, counter(4),  (gesamtZeit + timeCounter -55), endzeiten4, startzeiten4, autos_spur1_flag);}
  (junction 2833) -> (junction 2839) : {wartezeit_spur4_ges = gesamt_wartezeit_pro_spur(wartezeiten4, wartezeit_spur4_ges, alte_counter(4), counter(4));}
  (junction 3128) -> (junction 3143) : {[anz_autos4, autos_auf_spur4, counter(4), endzeiten4] = generiere_gruenphase(4, 55, autos_auf_spur4, counter(4),  (gesamtZeit + timeCounter -55), endzeiten4, startzeiten4, autos_spur1_flag);}
  (junction 2837) -> ampel2_rot14 : {gesamte_autos = berechne_gesamte_autos(counter(1), counter(2), counter(3), counter(4), counter(5), counter(6), counter(7));}
  (junction 1137) -> (junction 1147) : {[anz_autos4, autos_auf_spur4, counter(4), endzeiten4] = generiere_gruenphase(4, 75, autos_auf_spur4, counter(4),  (gesamtZeit + timeCounter - 75), endzeiten4, startzeiten4, autos_spur1_flag);}
  (junction 3142) -> (junction 3145) : {gesamtwartezeit = berechne_gesamtwartezeit(wartezeit_spur1_ges, wartezeit_spur2_ges, wartezeit_spur3_ges, wartezeit_spur4_ges, wartezeit_spur5_ges, wartezeit_spur6_ges, wartezeit_spur7_ges);}
  (junction 2841) -> (junction 2840) : {gesamtwartezeit = berechne_gesamtwartezeit(wartezeit_spur1_ges, wartezeit_spur2_ges, wartezeit_spur3_ges, wartezeit_spur4_ges, wartezeit_spur5_ges, wartezeit_spur6_ges, wartezeit_spur7_ges);}
  (junction 2838) -> ampel2_rot10 : {gesamte_autos = berechne_gesamte_autos(counter(1), counter(2), counter(3), counter(4), counter(5), counter(6), counter(7));}
  (junction 3131) -> (junction 3154) : {wartezeiten4 = berechne_wartezeiten(startzeiten4, endzeiten4, alte_counter(4), counter(4), wartezeiten4);}
  (junction 3129) -> (junction 3155) : {gesamtwartezeit = berechne_gesamtwartezeit(wartezeit_spur1_ges, wartezeit_spur2_ges, wartezeit_spur3_ges, wartezeit_spur4_ges, wartezeit_spur5_ges, wartezeit_spur6_ges, wartezeit_spur7_ges);}
  (junction 2839) -> (junction 2842) : {gesamtwartezeit = berechne_gesamtwartezeit(wartezeit_spur1_ges, wartezeit_spur2_ges, wartezeit_spur3_ges, wartezeit_spur4_ges, wartezeit_spur5_ges, wartezeit_spur6_ges, wartezeit_spur7_ges);}
  (junction 1747) -> (junction 1759) : {wartezeiten3 = berechne_wartezeiten(startzeiten3, endzeiten3, alte_counter(3), counter(3), wartezeiten3);}
  (junction 1144) -> (junction 1156) : {gesamtwartezeit = berechne_gesamtwartezeit(wartezeit_spur1_ges, wartezeit_spur2_ges, wartezeit_spur3_ges, wartezeit_spur4_ges, wartezeit_spur5_ges, wartezeit_spur6_ges, wartezeit_spur7_ges);}
  (junction 3143) -> (junction 3132) : {wartezeiten4 = berechne_wartezeiten(startzeiten4, endzeiten4, alte_counter(4), counter(4), wartezeiten4);}
  (junction 1147) -> (junction 1146) : {wartezeiten4 = berechne_wartezeiten(startzeiten4, endzeiten4, alte_counter(4), counter(4), wartezeiten4);}
  (junction 2840) -> ampel2_rot15 : {gesamte_autos = berechne_gesamte_autos(counter(1), counter(2), counter(3), counter(4), counter(5), counter(6), counter(7));}
  (junction 3145) -> (junction 3157) : {gesamte_autos = berechne_gesamte_autos(counter(1), counter(2), counter(3), counter(4), counter(5), counter(6), counter(7));}
  (junction 2842) -> ampel2_rot8 : {gesamte_autos = berechne_gesamte_autos(counter(1), counter(2), counter(3), counter(4), counter(5), counter(6), counter(7));}
  (junction 3155) -> (junction 3146) : {gesamte_autos = berechne_gesamte_autos(counter(1), counter(2), counter(3), counter(4), counter(5), counter(6), counter(7));}
  (junction 3154) -> (junction 3144) : {wartezeit_spur4_ges = gesamt_wartezeit_pro_spur(wartezeiten4, wartezeit_spur4_ges, alte_counter(4), counter(4));}
  (junction 3157) -> (junction 3149) : {[anz_autos4, autos_auf_spur4, counter(4), endzeiten4] = generiere_gruenphase(4, 42, autos_auf_spur4, counter(4),  (gesamtZeit + timeCounter -42), endzeiten4, startzeiten4, auslastung, autos_spur1_flag);}
  (junction 1156) -> (junction 1148) : {gesamte_autos = berechne_gesamte_autos(counter(1), counter(2), counter(3), counter(4), counter(5), counter(6), counter(7));}
  (junction 1759) -> (junction 1756) : {wartezeit_spur3_ges = gesamt_wartezeit_pro_spur(wartezeiten3, wartezeit_spur3_ges, alte_counter(3), counter(3));}
  ampel2_rot14 -> (junction 2835) : after(1,sec)
      | {timeCounter = refresher(timeCounter, 1);}
  (junction 3132) -> (junction 3159) : {wartezeit_spur4_ges = gesamt_wartezeit_pro_spur(wartezeiten4, wartezeit_spur4_ges, alte_counter(4), counter(4));}
  (junction 3146) -> (junction 3148) : {[anz_autos4, autos_auf_spur4, counter(4), endzeiten4] = generiere_gruenphase(4, 42, autos_auf_spur4, counter(4),  (gesamtZeit + timeCounter -42), endzeiten4, startzeiten4, auslastung, autos_spur1_flag);}
  (junction 1146) -> (junction 1149) : {wartezeit_spur4_ges = gesamt_wartezeit_pro_spur(wartezeiten4, wartezeit_spur4_ges, alte_counter(4), counter(4));}
  (junction 1148) -> (junction 1155) : {[anz_autos4, autos_auf_spur4, counter(4), endzeiten4] = generiere_gruenphase(4, 62, autos_auf_spur4, counter(4),  (gesamtZeit + timeCounter - 62), endzeiten4, startzeiten4, auslastung, autos_spur1_flag);}
  ampel2_rot10 -> (junction 2836) : after(1,sec)
      | {timeCounter = refresher(timeCounter, 1);}
  ampel2_rot6 -> (junction 1737) : {[anz_autos3, autos_auf_spur3, counter(3), endzeiten3] = generiere_gruenphase(3, 52, autos_auf_spur3, counter(3),  (gesamtZeit + timeCounter - 52), endzeiten3, startzeiten3, auslastung, autos_spur1_flag);}
  (junction 3149) -> (junction 3133) : {wartezeiten4 = berechne_wartezeiten(startzeiten4, endzeiten4, alte_counter(4), counter(4), wartezeiten4);}
  ampel2_rot15 -> (junction 2846) : after(1,sec)
      | {timeCounter = refresher(timeCounter, 1);}
  (junction 2835) -> rg3_rotgelb7 : {timer_spuren = countOnwards(timer_spuren,1,[1 1 1 1 1 1 1]);}
  (junction 3148) -> (junction 3158) : {wartezeiten4 = berechne_wartezeiten(startzeiten4, endzeiten4, alte_counter(4), counter(4), wartezeiten4);}
  ampel2_rot8 -> (junction 2843) : after(1,sec)
      | {timeCounter = refresher(timeCounter, 1);}
  (junction 3144) -> (junction 3138) : {gesamtwartezeit = berechne_gesamtwartezeit(wartezeit_spur1_ges, wartezeit_spur2_ges, wartezeit_spur3_ges, wartezeit_spur4_ges, wartezeit_spur5_ges, wartezeit_spur6_ges, wartezeit_spur7_ges);}
  (junction 1155) -> (junction 1140) : {wartezeiten4 = berechne_wartezeiten(startzeiten4, endzeiten4, alte_counter(4), counter(4), wartezeiten4);}
  (junction 2836) -> rg3_rotgelb4 : {timer_spuren = countOnwards(timer_spuren,1,[1 1 1 1 1 1 1]);}
  (junction 1756) -> (junction 1740) : {gesamtwartezeit = berechne_gesamtwartezeit(wartezeit_spur1_ges, wartezeit_spur2_ges, wartezeit_spur3_ges, wartezeit_spur4_ges, wartezeit_spur5_ges, wartezeit_spur6_ges, wartezeit_spur7_ges);}
  (junction 2846) -> rg3_rotgelb8 : {timer_spuren = countOnwards(timer_spuren,1,[1 1 1 1 1 1 1]);}
  (junction 1737) -> (junction 1761) : {wartezeiten3 = berechne_wartezeiten(startzeiten3, endzeiten3, alte_counter(3), counter(3), wartezeiten3);}
  (junction 3159) -> (junction 3141) : {gesamtwartezeit = berechne_gesamtwartezeit(wartezeit_spur1_ges, wartezeit_spur2_ges, wartezeit_spur3_ges, wartezeit_spur4_ges, wartezeit_spur5_ges, wartezeit_spur6_ges, wartezeit_spur7_ges);}
  (junction 3133) -> (junction 3130) : {wartezeit_spur4_ges = gesamt_wartezeit_pro_spur(wartezeiten4, wartezeit_spur4_ges, alte_counter(4), counter(4));}
  (junction 2843) -> rg3_rotgelb5 : {timer_spuren = countOnwards(timer_spuren,1,[1 1 1 1 1 1 1]);}
  (junction 1149) -> (junction 1157) : {gesamtwartezeit = berechne_gesamtwartezeit(wartezeit_spur1_ges, wartezeit_spur2_ges, wartezeit_spur3_ges, wartezeit_spur4_ges, wartezeit_spur5_ges, wartezeit_spur6_ges, wartezeit_spur7_ges);}
  rg3_rotgelb7 -> (junction 2845)
  (junction 3158) -> (junction 3134) : {wartezeit_spur4_ges = gesamt_wartezeit_pro_spur(wartezeiten4, wartezeit_spur4_ges, alte_counter(4), counter(4));}
  rg3_rotgelb4 -> (junction 2655)
  (junction 1140) -> (junction 1136) : {wartezeit_spur4_ges = gesamt_wartezeit_pro_spur(wartezeiten4, wartezeit_spur4_ges, alte_counter(4), counter(4));}
  (junction 3138) -> ampel2_rot16 : {gesamte_autos = berechne_gesamte_autos(counter(1), counter(2), counter(3), counter(4), counter(5), counter(6), counter(7));}
  (junction 1740) -> (junction 1749) : {gesamte_autos = berechne_gesamte_autos(counter(1), counter(2), counter(3), counter(4), counter(5), counter(6), counter(7));}
  rg3_rotgelb8 -> (junction 2847)
  (junction 3130) -> (junction 3135) : {gesamtwartezeit = berechne_gesamtwartezeit(wartezeit_spur1_ges, wartezeit_spur2_ges, wartezeit_spur3_ges, wartezeit_spur4_ges, wartezeit_spur5_ges, wartezeit_spur6_ges, wartezeit_spur7_ges);}
  (junction 3141) -> ampel2_rot22 : {gesamte_autos = berechne_gesamte_autos(counter(1), counter(2), counter(3), counter(4), counter(5), counter(6), counter(7));}
  (junction 2845) -> (junction 2844)
  (junction 2847) -> (junction 2845)
  rg3_rotgelb5 -> (junction 2678)
  (junction 1761) -> (junction 1750) : {wartezeit_spur3_ges = gesamt_wartezeit_pro_spur(wartezeiten3, wartezeit_spur3_ges, alte_counter(3), counter(3));}
  (junction 2844) -> (junction 2673)
  (junction 1157) -> ampel2_rot2 : {gesamte_autos = berechne_gesamte_autos(counter(1), counter(2), counter(3), counter(4), counter(5), counter(6), counter(7));}
  (junction 3134) -> (junction 3150) : {gesamtwartezeit = berechne_gesamtwartezeit(wartezeit_spur1_ges, wartezeit_spur2_ges, wartezeit_spur3_ges, wartezeit_spur4_ges, wartezeit_spur5_ges, wartezeit_spur6_ges, wartezeit_spur7_ges);}
  (junction 2655) -> (junction 2677)
  (junction 2678) -> (junction 2655)
  (junction 2677) -> (junction 2656)
  (junction 1136) -> (junction 1141) : {gesamtwartezeit = berechne_gesamtwartezeit(wartezeit_spur1_ges, wartezeit_spur2_ges, wartezeit_spur3_ges, wartezeit_spur4_ges, wartezeit_spur5_ges, wartezeit_spur6_ges, wartezeit_spur7_ges);}
  (junction 3135) -> ampel2_rot18 : {gesamte_autos = berechne_gesamte_autos(counter(1), counter(2), counter(3), counter(4), counter(5), counter(6), counter(7));}
  (junction 1749) -> (junction 1752) : {[anz_autos4, autos_auf_spur4, counter(4), endzeiten4] = generiere_gruenphase(4, 65, autos_auf_spur4, counter(4),  (gesamtZeit + timeCounter - 65), endzeiten4, startzeiten4, autos_spur1_flag);}
  (junction 3150) -> ampel2_rot23 : {gesamte_autos = berechne_gesamte_autos(counter(1), counter(2), counter(3), counter(4), counter(5), counter(6), counter(7));}
  (junction 1141) -> ampel2_rot3 : {gesamte_autos = berechne_gesamte_autos(counter(1), counter(2), counter(3), counter(4), counter(5), counter(6), counter(7));}
  (junction 1750) -> (junction 1763) : {gesamtwartezeit = berechne_gesamtwartezeit(wartezeit_spur1_ges, wartezeit_spur2_ges, wartezeit_spur3_ges, wartezeit_spur4_ges, wartezeit_spur5_ges, wartezeit_spur6_ges, wartezeit_spur7_ges);}
  ampel2_rot16 -> (junction 3137) : after(1,sec)
      | {timeCounter = refresher(timeCounter, 1);}
  (junction 1752) -> (junction 1766) : {wartezeiten4 = berechne_wartezeiten(startzeiten4, endzeiten4, alte_counter(4), counter(4), wartezeiten4);}
  ampel2_rot22 -> (junction 3170) : after(1,sec)
      | {timeCounter = refresher(timeCounter, 1);}
  ampel2_rot18 -> (junction 3151) : after(1,sec)
      | {timeCounter = refresher(timeCounter, 1);}
  ampel2_rot2 -> (junction 1142) : after(1,sec)
      | {timeCounter = refresher(timeCounter, 1);}
  (junction 3137) -> rg3_rotgelb10 : {timer_spuren = countOnwards(timer_spuren,1,[1 1 1 1 1 1 1]);}
  (junction 1763) -> (junction 1745) : {gesamte_autos = berechne_gesamte_autos(counter(1), counter(2), counter(3), counter(4), counter(5), counter(6), counter(7));}
  ampel2_rot23 -> (junction 3174) : after(1,sec)
      | {timeCounter = refresher(timeCounter, 1);}
  ampel2_rot3 -> (junction 1163) : after(1,sec)
      | {timeCounter = refresher(timeCounter, 1);}
  (junction 3151) -> rg3_rotgelb12 : {timer_spuren = countOnwards(timer_spuren,1,[1 1 1 1 1 1 1]);}
  (junction 3170) -> rg3_rotgelb11 : {timer_spuren = countOnwards(timer_spuren,1,[1 1 1 1 1 1 1]);}
  (junction 1766) -> (junction 1754) : {wartezeit_spur4_ges = gesamt_wartezeit_pro_spur(wartezeiten4, wartezeit_spur4_ges, alte_counter(4), counter(4));}
  (junction 1745) -> (junction 1736) : {[anz_autos4, autos_auf_spur4, counter(4), endzeiten4] = generiere_gruenphase(4, 52, autos_auf_spur4, counter(4),  (gesamtZeit + timeCounter - 52), endzeiten4, startzeiten4, auslastung, autos_spur1_flag);}
  (junction 1142) -> rg3_rotgelb : {timer_spuren = countOnwards(timer_spuren,1,[1 1 1 1 1 1 1]);}
  (junction 3174) -> rg3_rotgelb9 : {timer_spuren = countOnwards(timer_spuren,1,[1 1 1 1 1 1 1]);}
  rg3_rotgelb10 -> (junction 3183)
  (junction 1163) -> rg3_rotgelb1 : {timer_spuren = countOnwards(timer_spuren,1,[1 1 1 1 1 1 1]);}
  (junction 2656) -> (junction 2659)
  (junction 2673) -> (junction 2656)
  rg3_rotgelb11 -> (junction 3172)
  (junction 2659) -> (junction 2660) : {[autos_auf_spur5, spur5] = autos_auf_spur_generieren(spur5, gesamtZeit + timeCounter, autos_auf_spur5);}
  (junction 1736) -> (junction 1755) : {wartezeiten4 = berechne_wartezeiten(startzeiten4, endzeiten4, alte_counter(4), counter(4), wartezeiten4);}
  rg3_rotgelb12 -> (junction 3171)
  rg3_rotgelb -> (junction 1133)
  (junction 3183) -> (junction 3176)
  (junction 3171) -> (junction 3183)
  (junction 3176) -> (junction 3161)
  rg3_rotgelb9 -> (junction 3175)
  (junction 1754) -> (junction 1777) : {gesamtwartezeit = berechne_gesamtwartezeit(wartezeit_spur1_ges, wartezeit_spur2_ges, wartezeit_spur3_ges, wartezeit_spur4_ges, wartezeit_spur5_ges, wartezeit_spur6_ges, wartezeit_spur7_ges);}
  rg3_rotgelb1 -> (junction 1150)
  (junction 3172) -> (junction 3184)
  (junction 3175) -> (junction 3172)
  (junction 3184) -> (junction 3166)
  (junction 1133) -> (junction 1138)
  (junction 1150) -> (junction 1133)
  (junction 1755) -> (junction 1769) : {wartezeit_spur4_ges = gesamt_wartezeit_pro_spur(wartezeiten4, wartezeit_spur4_ges, alte_counter(4), counter(4));}
  (junction 1138) -> (junction 1151) : {[autos_auf_spur5, spur5] = autos_auf_spur_generieren(spur5, gesamtZeit + timeCounter, autos_auf_spur5);}
  (junction 1777) -> ampel2_rot7 : {gesamte_autos = berechne_gesamte_autos(counter(1), counter(2), counter(3), counter(4), counter(5), counter(6), counter(7));}
  (junction 1769) -> (junction 1791) : {gesamtwartezeit = berechne_gesamtwartezeit(wartezeit_spur1_ges, wartezeit_spur2_ges, wartezeit_spur3_ges, wartezeit_spur4_ges, wartezeit_spur5_ges, wartezeit_spur6_ges, wartezeit_spur7_ges);}
  (junction 1791) -> ampel2_rot4 : {gesamte_autos = berechne_gesamte_autos(counter(1), counter(2), counter(3), counter(4), counter(5), counter(6), counter(7));}
  (junction 1151) -> (junction 1154) [order 1] : [autos_auf_spur5 == 0]
  (junction 1151) -> (junction 1139) [order 2]
  (junction 1154) -> (junction 1160) : after(1,sec)
      | {timeCounter = refresher(timeCounter, 1);}
  (junction 3161) -> (junction 3186)
  (junction 3166) -> (junction 3161)
  (junction 3186) -> (junction 3177) : {[autos_auf_spur5, spur5] = autos_auf_spur_generieren(spur5, gesamtZeit + timeCounter, autos_auf_spur5);}
  ampel2_rot7 -> (junction 1775) : after(1,sec)
      | {timeCounter = refresher(timeCounter, 1);}
  (junction 1139) -> (junction 1159) [order 1] : [autos_auf_spur5 > 0]
  (junction 1139) -> (junction 1184) [order 2]
  (junction 1159) -> l3_rotgelb_rg3_fuss6_gruen
  ampel2_rot4 -> (junction 1799) : after(1,sec)
      | {timeCounter = refresher(timeCounter, 1);}
  (junction 1775) -> rg3_rotgelb2 : {timer_spuren = countOnwards(timer_spuren,1,[1 1 1 1 1 1 1]);}
  (junction 1160) -> rg3_fuss6_gruen : {timer_spuren = countOnwards(timer_spuren,1,[1 1 1 1 1 1 1]);}
  (junction 1799) -> rg3_rotgelb3 : {timer_spuren = countOnwards(timer_spuren,1,[1 1 1 1 1 1 1]);}
  rg3_rotgelb2 -> (junction 1776)
  rg3_rotgelb3 -> (junction 1792)
  (junction 1776) -> (junction 1768)
  (junction 1792) -> (junction 1776)
  l3_rotgelb_rg3_fuss6_gruen -> (junction 1162) : {[autos_auf_spur6, spur6] = autos_auf_spur_generieren(spur6, gesamtZeit + timeCounter, autos_auf_spur6);}
  rg3_fuss6_gruen -> (junction 1132) : {[autos_auf_spur6, spur6] = autos_auf_spur_generieren(spur6, gesamtZeit + timeCounter, autos_auf_spur6);}
  (junction 1768) -> (junction 1783) : {[autos_auf_spur5, spur5] = autos_auf_spur_generieren(spur5, gesamtZeit + timeCounter, autos_auf_spur5);}
  (junction 1132) -> (junction 1161) : after(4,sec)
      | {timeCounter = refresher(timeCounter, 4);}
  (junction 1162) -> (junction 1152) : after(1,sec)
      | {timeCounter = refresher(timeCounter, 1);}
  (junction 1152) -> l3_gruen : {timer_spuren = countOnwards(timer_spuren,1,[1 1 1 1 1 0 1]);}
  (junction 1161) -> ampel4_rotgelb : {timer_spuren = countOnwards(timer_spuren,4,[1 1 1 1 1 0 1]);}
  (junction 1783) -> (junction 1770) [order 1] : [autos_auf_spur5 == 0]
  (junction 1783) -> (junction 1797) [order 2]
  (junction 1770) -> (junction 1767) : after(1,sec)
      | {timeCounter = refresher(timeCounter, 1);}
  (junction 2660) -> rg3_rotgelb6 [order 1] : [autos_auf_spur5 == 0]
  (junction 2660) -> (junction 2671) [order 2]
  ampel4_rotgelb -> (junction 1134) : after(1,sec)
      | {timeCounter = refresher(timeCounter, 1);}
  rg3_rotgelb6 -> (junction 2668) : after(1,sec)
      | {timeCounter = refresher(timeCounter, 1);}
  (junction 1797) -> (junction 1793) [order 1] : [autos_auf_spur5 > 0]
  (junction 1797) -> (junction 1800) [order 2]
  (junction 1793) -> l3_rotgelb_rg3_fuss6_gruen1
  (junction 2671) -> (junction 2667) [order 1] : [autos_auf_spur5 > 0]
  (junction 2671) -> (junction 2470) [order 2]
  l3_gruen -> (junction 1135) : after(8,sec)
      | {timeCounter = refresher(timeCounter, 8);}
  (junction 2667) -> l3_rotgelb_rg3_fuss6_gruen2
  (junction 1767) -> rg3_fuss6_gruen1 : {timer_spuren = countOnwards(timer_spuren,1,[1 1 1 1 1 1 1]);}
  (junction 2668) -> rg3_fuss6_gruen2 : {timer_spuren = countOnwards(timer_spuren,1,[1 1 1 1 1 1 1]);}
  (junction 1134) -> ampel4_fuss5_gruen : {timer_spuren = countOnwards(timer_spuren,1,[1 1 1 1 1 0 1]);}
  (junction 1135) -> l3_gelb : {timer_spuren = countOnwards(timer_spuren,8,[1 1 1 1 0 0 1]);}
  l3_rotgelb_rg3_fuss6_gruen1 -> (junction 1794) : {[autos_auf_spur6, spur6] = autos_auf_spur_generieren(spur6, gesamtZeit + timeCounter, autos_auf_spur6);}
  rg3_fuss6_gruen1 -> (junction 1771) : {[autos_auf_spur6, spur6] = autos_auf_spur_generieren(spur6, gesamtZeit + timeCounter, autos_auf_spur6);}
  l3_rotgelb_rg3_fuss6_gruen2 -> (junction 2674) : {[autos_auf_spur6, spur6] = autos_auf_spur_generieren(spur6, gesamtZeit + timeCounter, autos_auf_spur6);}
  rg3_fuss6_gruen2 -> (junction 2676) : {[autos_auf_spur6, spur6] = autos_auf_spur_generieren(spur6, gesamtZeit + timeCounter, autos_auf_spur6);}
  (junction 1771) -> (junction 1784) : after(4,sec)
      | {timeCounter = refresher(timeCounter, 4);}
  (junction 1794) -> (junction 1786) : after(1,sec)
      | {timeCounter = refresher(timeCounter, 1);}
  (junction 3177) -> (junction 3182) [order 1] : [autos_auf_spur5 == 0]
  (junction 2676) -> (junction 2658) : after(4,sec)
      | {timeCounter = refresher(timeCounter, 4);}
  (junction 3177) -> (junction 3173) [order 2]
  (junction 3182) -> (junction 3178) : after(1,sec)
      | {timeCounter = refresher(timeCounter, 1);}
  (junction 2674) -> (junction 2661) : after(1,sec)
      | {timeCounter = refresher(timeCounter, 1);}
  (junction 1786) -> l3_gruen1 : {timer_spuren = countOnwards(timer_spuren,1,[1 1 1 1 1 0 1]);}
  (junction 1784) -> ampel4_rotgelb1 : {timer_spuren = countOnwards(timer_spuren,4,[1 1 1 1 1 0 1]);}
  (junction 3173) -> (junction 3187) [order 1] : [autos_auf_spur5 > 0]
  (junction 3173) -> (junction 3203) [order 2]
  (junction 3187) -> l3_rotgelb_rg3_fuss6_gruen3
  l3_gelb -> (junction 1145) : after(3,sec)
      | {timeCounter = refresher(timeCounter, 3);}
  (junction 2661) -> l3_gruen2 : {timer_spuren = countOnwards(timer_spuren,1,[1 1 1 1 1 0 1]);}
  (junction 2658) -> ampel4_rotgelb2 : {timer_spuren = countOnwards(timer_spuren,4,[1 1 1 1 1 0 1]);}
  (junction 3178) -> rg3_fuss6_gruen3 : {timer_spuren = countOnwards(timer_spuren,1,[1 1 1 1 1 1 1]);}
  (junction 1145) -> (junction 1172) : {timer_spuren = countOnwards(timer_spuren,3,[1 1 1 1 0 0 1]);}
  ampel4_rotgelb1 -> (junction 1787) : after(1,sec)
      | {timeCounter = refresher(timeCounter, 1);}
  ampel4_rotgelb2 -> (junction 2675) : after(1,sec)
      | {timeCounter = refresher(timeCounter, 1);}
  l3_gruen1 -> (junction 1795) : after(8,sec)
      | {timeCounter = refresher(timeCounter, 8);}
  (junction 1172) -> l3_fuss6_rot : {[autos_auf_spur5, spur5] = autos_auf_spur_generieren(spur5, gesamtZeit + timeCounter, autos_auf_spur5);}
  l3_gruen2 -> (junction 2657) : after(6,sec)
      | {timeCounter = refresher(timeCounter, 6);}
  ampel4_fuss5_gruen -> (junction 1190) : {[autos_auf_spur7, spur7] = autos_auf_spur_generieren(spur7, gesamtZeit + timeCounter, autos_auf_spur7);}
  l3_rotgelb_rg3_fuss6_gruen3 -> (junction 3160) : {[autos_auf_spur6, spur6] = autos_auf_spur_generieren(spur6, gesamtZeit + timeCounter, autos_auf_spur6);}
  rg3_fuss6_gruen3 -> (junction 3167) : {[autos_auf_spur6, spur6] = autos_auf_spur_generieren(spur6, gesamtZeit + timeCounter, autos_auf_spur6);}
  (junction 1787) -> ampel4_fuss5_gruen2 : {timer_spuren = countOnwards(timer_spuren,1,[1 1 1 1 1 0 1]);}
  (junction 1190) -> (junction 1176) : after(6,sec)
      | {timeCounter = refresher(timeCounter, 6);}
  (junction 3167) -> (junction 3168) : after(4,sec)
      | {timeCounter = refresher(timeCounter, 4);}
  (junction 2675) -> ampel4_fuss5_gruen4 : {timer_spuren = countOnwards(timer_spuren,1,[1 1 1 1 1 0 1]);}
  (junction 1795) -> l3_gelb1 : {timer_spuren = countOnwards(timer_spuren,8,[1 1 1 1 0 0 1]);}
  (junction 3160) -> (junction 3162) : after(1,sec)
      | {timeCounter = refresher(timeCounter, 1);}
  (junction 2657) -> l3_gelb_fuss6_rot : {timer_spuren = countOnwards(timer_spuren,6,[1 1 1 1 0 0 1]);}
  l3_fuss6_rot -> (junction 1171) : {[anz_autos5, autos_auf_spur5, counter(5), endzeiten5] = generiere_gruenphase(5, 11, autos_auf_spur5, counter(5),  (gesamtZeit + timeCounter -11), endzeiten5, startzeiten5, auslastung, autos_spur1_flag);}
  (junction 3162) -> l3_gruen3 : {timer_spuren = countOnwards(timer_spuren,1,[1 1 1 1 1 0 1]);}
  (junction 3168) -> ampel4_rotgelb3 : {timer_spuren = countOnwards(timer_spuren,4,[1 1 1 1 1 0 1]);}
  ampel4_rotgelb3 -> (junction 3185) : after(1,sec)
      | {timeCounter = refresher(timeCounter, 1);}
  (junction 1171) -> (junction 1193) : {wartezeiten5 = berechne_wartezeiten(startzeiten5, endzeiten5, alte_counter(5), counter(5), wartezeiten5);}
  l3_gelb_fuss6_rot -> (junction 2666) : after(1,sec)
      | {timeCounter = refresher(timeCounter, 1);}
  l3_gelb1 -> (junction 1798) : after(3,sec)
      | {timeCounter = refresher(timeCounter, 3);}
  l3_gruen3 -> (junction 3180) : after(3,sec)
      | {timeCounter = refresher(timeCounter, 3);}
  (junction 2666) -> (junction 2672) : {timer_spuren = countOnwards(timer_spuren,1,[1 1 1 1 0 0 1]);}
  (junction 1798) -> (junction 1785) : {timer_spuren = countOnwards(timer_spuren,3,[1 1 1 1 0 0 1]);}
  (junction 1193) -> (junction 1166) : {wartezeit_spur5_ges = gesamt_wartezeit_pro_spur(wartezeiten5, wartezeit_spur5_ges, alte_counter(5), counter(5));}
  (junction 3185) -> ampel4_fuss5_gruen6 : {timer_spuren = countOnwards(timer_spuren,1,[1 1 1 1 1 0 1]);}
  (junction 2672) -> fuss6_rot2 : {[autos_auf_spur5, spur5] = autos_auf_spur_generieren(spur5, gesamtZeit + timeCounter, autos_auf_spur5);}
  (junction 1785) -> l3_fuss6_rot3 : {[autos_auf_spur5, spur5] = autos_auf_spur_generieren(spur5, gesamtZeit + timeCounter, autos_auf_spur5);}
  (junction 3180) -> l3_gelb2 : {timer_spuren = countOnwards(timer_spuren,3,[1 1 1 1 0 0 1]);}
  ampel4_fuss5_gruen2 -> (junction 1772) : {[autos_auf_spur7, spur7] = autos_auf_spur_generieren(spur7, gesamtZeit + timeCounter, autos_auf_spur7);}
  ampel4_fuss5_gruen4 -> (junction 2662) : {[autos_auf_spur7, spur7] = autos_auf_spur_generieren(spur7, gesamtZeit + timeCounter, autos_auf_spur7);}
  (junction 1166) -> (junction 1164) : {gesamtwartezeit = berechne_gesamtwartezeit(wartezeit_spur1_ges, wartezeit_spur2_ges, wartezeit_spur3_ges, wartezeit_spur4_ges, wartezeit_spur5_ges, wartezeit_spur6_ges, wartezeit_spur7_ges);}
  fuss6_rot2 -> (junction 2663) : after(2,sec)
      | {timeCounter = refresher(timeCounter, 2);}
  (junction 1772) -> (junction 1780) : after(6,sec)
      | {timeCounter = refresher(timeCounter, 6);}
  (junction 1164) -> l3_fuss6_rot1 : {gesamte_autos = berechne_gesamte_autos(counter(1), counter(2), counter(3), counter(4), counter(5), counter(6), counter(7));}
  (junction 2662) -> (junction 2456) : after(2,sec)
      | {timeCounter = refresher(timeCounter, 2);}
  l3_fuss6_rot3 -> (junction 1796) : {[anz_autos5, autos_auf_spur5, counter(5), endzeiten5] = generiere_gruenphase(5, 11, autos_auf_spur5, counter(5),  (gesamtZeit + timeCounter -11), endzeiten5, startzeiten5, auslastung, autos_spur1_flag);}
  (junction 2663) -> l3_rot1 : {timer_spuren = countOnwards(timer_spuren,2,[1 1 1 1 0 0 1]);}
  (junction 1176) -> fuss6_rot : {timer_spuren = countOnwards(timer_spuren,6,[1 1 1 1 1 0 0]);}
  l3_gelb2 -> fuss6_rot4 : after(1,sec)
      | {timeCounter = refresher(timeCounter, 1);}
  l3_rot1 -> (junction 2664) : {[anz_autos5, autos_auf_spur5, counter(5), endzeiten5] = generiere_gruenphase(5, 9, autos_auf_spur5, counter(5),  (gesamtZeit + timeCounter - 9), endzeiten5, startzeiten5, auslastung, autos_spur1_flag);}
  l3_fuss6_rot1 -> (junction 1179) : after(2,sec)
      | {timeCounter = refresher(timeCounter, 2);}
  (junction 1796) -> (junction 1773) : {wartezeiten5 = berechne_wartezeiten(startzeiten5, endzeiten5, alte_counter(5), counter(5), wartezeiten5);}
  fuss6_rot -> (junction 1186) : after(2,sec)
      | {timeCounter = refresher(timeCounter, 2);}
  (junction 2664) -> (junction 2669) : {wartezeiten5 = berechne_wartezeiten(startzeiten5, endzeiten5, alte_counter(5), counter(5), wartezeiten5);}
  fuss6_rot4 -> (junction 3163) : after(2,sec)
      | {timeCounter = refresher(timeCounter, 2);}
  (junction 1179) -> rg3_gelb1 : {timer_spuren = countOnwards(timer_spuren,2,[1 1 1 1 1 0 1]);}
  ampel4_fuss5_gruen6 -> fuss6_rot5 : {[autos_auf_spur7, spur7] = autos_auf_spur_generieren(spur7, gesamtZeit + timeCounter, autos_auf_spur7);}
  (junction 1186) -> rg3_gelb : {timer_spuren = countOnwards(timer_spuren,2,[1 1 1 1 1 0 0]);}
  (junction 1773) -> (junction 1774) : {wartezeit_spur5_ges = gesamt_wartezeit_pro_spur(wartezeiten5, wartezeit_spur5_ges, alte_counter(5), counter(5));}
  (junction 3163) -> (junction 3164) : {timer_spuren = countOnwards(timer_spuren,3,[1 1 1 1 0 0 1]);}
  (junction 2669) -> (junction 2665) : {wartezeit_spur5_ges = gesamt_wartezeit_pro_spur(wartezeiten5, wartezeit_spur5_ges, alte_counter(5), counter(5));}
  (junction 3164) -> l3_rot_rg3_gelb : {[autos_auf_spur5, spur5] = autos_auf_spur_generieren(spur5, gesamtZeit + timeCounter, autos_auf_spur5);}
  rg3_gelb1 -> (junction 1169) : after(3,sec)
      | {timeCounter = refresher(timeCounter, 3);}
  rg3_gelb -> (junction 1188) : after(3,sec)
      | {timeCounter = refresher(timeCounter, 3);}
  (junction 1774) -> (junction 1779) : {gesamtwartezeit = berechne_gesamtwartezeit(wartezeit_spur1_ges, wartezeit_spur2_ges, wartezeit_spur3_ges, wartezeit_spur4_ges, wartezeit_spur5_ges, wartezeit_spur6_ges, wartezeit_spur7_ges);}
  (junction 2665) -> (junction 2670) : {gesamtwartezeit = berechne_gesamtwartezeit(wartezeit_spur1_ges, wartezeit_spur2_ges, wartezeit_spur3_ges, wartezeit_spur4_ges, wartezeit_spur5_ges, wartezeit_spur6_ges, wartezeit_spur7_ges);}
  (junction 1779) -> l3_fuss6_rot2 : {gesamte_autos = berechne_gesamte_autos(counter(1), counter(2), counter(3), counter(4), counter(5), counter(6), counter(7));}
  (junction 1169) -> (junction 1189) : {timer_spuren = countOnwards(timer_spuren,3,[1 1 1 1 1 0 1]);}
  l3_rot_rg3_gelb -> (junction 3165) : {[anz_autos5, autos_auf_spur5, counter(5), endzeiten5] = generiere_gruenphase(5, 6, autos_auf_spur5, counter(5),  (gesamtZeit + timeCounter - 6), endzeiten5, startzeiten5, auslastung, autos_spur1_flag);}
  (junction 2670) -> l3_rot : {gesamte_autos = berechne_gesamte_autos(counter(1), counter(2), counter(3), counter(4), counter(5), counter(6), counter(7));}
  (junction 1188) -> (junction 1194) : {timer_spuren = countOnwards(timer_spuren,3,[1 1 1 1 1 0 0]);}
  (junction 1780) -> fuss6_rot1 : {timer_spuren = countOnwards(timer_spuren,6,[1 1 1 1 1 0 0]);}
  (junction 3165) -> (junction 3190) : {wartezeiten5 = berechne_wartezeiten(startzeiten5, endzeiten5, alte_counter(5), counter(5), wartezeiten5);}
  (junction 1189) -> rg3_rot_ampel4_rotgelb : {[autos_auf_spur6, spur6] = autos_auf_spur_generieren(spur6, gesamtZeit + timeCounter, autos_auf_spur6);}
  (junction 2456) -> fuss6_rot3 : {timer_spuren = countOnwards(timer_spuren,2,[1 1 1 1 1 0 0]);}
  l3_rot -> (junction 2461) : %after(2,sec)
      | %{timeCounter = refresher(timeCounter, 2);}
  l3_fuss6_rot2 -> (junction 1778) : after(2,sec)
      | {timeCounter = refresher(timeCounter, 2);}
  (junction 3190) -> (junction 3179) : {wartezeit_spur5_ges = gesamt_wartezeit_pro_spur(wartezeiten5, wartezeit_spur5_ges, alte_counter(5), counter(5));}
  fuss6_rot1 -> (junction 1781) : after(2,sec)
      | {timeCounter = refresher(timeCounter, 2);}
  fuss6_rot3 -> (junction 2457) : after(2,sec)
      | {timeCounter = refresher(timeCounter, 2);}
  (junction 1778) -> rg3_gelb2 : {timer_spuren = countOnwards(timer_spuren,2,[1 1 1 1 1 0 1]);}
  (junction 1781) -> rg3_gelb3 : {timer_spuren = countOnwards(timer_spuren,2,[1 1 1 1 1 0 0]);}
  (junction 1194) -> rg3_fuss5_rot : {[autos_auf_spur6, spur6] = autos_auf_spur_generieren(spur6, gesamtZeit + timeCounter, autos_auf_spur6);}
  (junction 2461) -> rg3_gelb4 : %{timer_spuren = countOnwards(timer_spuren,2,[1 1 1 1 1 0 1]);}
  (junction 2457) -> rg3_gelb5 : {timer_spuren = countOnwards(timer_spuren,2,[1 1 1 1 1 0 0]);}
  (junction 3179) -> (junction 3188) : {gesamtwartezeit = berechne_gesamtwartezeit(wartezeit_spur1_ges, wartezeit_spur2_ges, wartezeit_spur3_ges, wartezeit_spur4_ges, wartezeit_spur5_ges, wartezeit_spur6_ges, wartezeit_spur7_ges);}
  rg3_rot_ampel4_rotgelb -> (junction 1192) : {[anz_autos6, autos_auf_spur6, counter(6), endzeiten6] = generiere_gruenphase(6, 17, autos_auf_spur6, counter(6),  (gesamtZeit + timeCounter -17), endzeiten6, startzeiten6, auslastung, autos_spur1_flag);}
  (junction 3188) -> l3_rot_rg3_gelb1 : {gesamte_autos = berechne_gesamte_autos(counter(1), counter(2), counter(3), counter(4), counter(5), counter(6), counter(7));}
  rg3_gelb2 -> (junction 1782) : after(3,sec)
      | {timeCounter = refresher(timeCounter, 3);}
  rg3_gelb3 -> (junction 1788) : after(3,sec)
      | {timeCounter = refresher(timeCounter, 3);}
  rg3_gelb4 -> (junction 2458) : after(3,sec)
      | {timeCounter = refresher(timeCounter, 3);}
  rg3_gelb5 -> (junction 2454) : after(3,sec)
      | {timeCounter = refresher(timeCounter, 3);}
  (junction 1782) -> (junction 1789) : {timer_spuren = countOnwards(timer_spuren,3,[1 1 1 1 1 0 1]);}
  (junction 1192) -> (junction 1182) : {wartezeiten6 = berechne_wartezeiten(startzeiten6, endzeiten6, alte_counter(6), counter(6), wartezeiten6);}
  (junction 2458) -> (junction 2459) : {timer_spuren = countOnwards(timer_spuren,3,[1 1 1 1 1 0 1]);}
  (junction 1788) -> (junction 1790) : {timer_spuren = countOnwards(timer_spuren,3,[1 1 1 1 1 0 0]);}
  rg3_fuss5_rot -> (junction 1185) : {[anz_autos6, autos_auf_spur6, counter(6), endzeiten6] = generiere_gruenphase(6, 17, autos_auf_spur6, counter(6),  (gesamtZeit + timeCounter -17), endzeiten6, startzeiten6, auslastung, autos_spur1_flag);}
  (junction 2454) -> (junction 2460) : {timer_spuren = countOnwards(timer_spuren,3,[1 1 1 1 1 0 0]);}
  (junction 1789) -> rg3_rot_ampel4_rotgelb2 : {[autos_auf_spur6, spur6] = autos_auf_spur_generieren(spur6, gesamtZeit + timeCounter, autos_auf_spur6);}
  fuss6_rot5 -> (junction 3181) : after(2,sec)
      | {timeCounter = refresher(timeCounter, 2);}
  (junction 2459) -> rg3_rot_ampel4_rotgelb4 : {[autos_auf_spur6, spur6] = autos_auf_spur_generieren(spur6, gesamtZeit + timeCounter, autos_auf_spur6);}
  (junction 1182) -> (junction 1177) : {wartezeit_spur6_ges = gesamt_wartezeit_pro_spur(wartezeiten6, wartezeit_spur6_ges, alte_counter(6), counter(6));}
  (junction 3181) -> rg3_gelb6 : {timer_spuren = countOnwards(timer_spuren,2,[1 1 1 1 1 0 0]);}
  l3_rot_rg3_gelb1 -> (junction 3189) : after(3,sec)
      | {timeCounter = refresher(timeCounter, 3);}
  (junction 1177) -> (junction 1191) : {gesamtwartezeit = berechne_gesamtwartezeit(wartezeit_spur1_ges, wartezeit_spur2_ges, wartezeit_spur3_ges, wartezeit_spur4_ges, wartezeit_spur5_ges, wartezeit_spur6_ges, wartezeit_spur7_ges);}
  (junction 1790) -> rg3_fuss5_rot2 : {[autos_auf_spur6, spur6] = autos_auf_spur_generieren(spur6, gesamtZeit + timeCounter, autos_auf_spur6);}
  rg3_gelb6 -> (junction 3169) : after(1,sec)
      | {timeCounter = refresher(timeCounter, 1);}
  (junction 2460) -> rg3_fuss5_rot5 : {[autos_auf_spur6, spur6] = autos_auf_spur_generieren(spur6, gesamtZeit + timeCounter, autos_auf_spur6);}
  rg3_rot_ampel4_rotgelb2 -> (junction 1826) : {[anz_autos6, autos_auf_spur6, counter(6), endzeiten6] = generiere_gruenphase(6, 17, autos_auf_spur6, counter(6),  (gesamtZeit + timeCounter -17), endzeiten6, startzeiten6, auslastung, autos_spur1_flag);}
  rg3_rot_ampel4_rotgelb4 -> (junction 2455) : {[anz_autos6, autos_auf_spur6, counter(6), endzeiten6] = generiere_gruenphase(6, 12, autos_auf_spur6, counter(6),  (gesamtZeit + timeCounter - 12), endzeiten6, startzeiten6, auslastung, autos_spur1_flag);}
  (junction 1191) -> rg3_rot_ampel4_rotgelb1 : {gesamte_autos = berechne_gesamte_autos(counter(1), counter(2), counter(3), counter(4), counter(5), counter(6), counter(7));}
  (junction 3189) -> (junction 3214) : {timer_spuren = countOnwards(timer_spuren,3,[1 1 1 1 1 0 1]);}
  (junction 1185) -> (junction 1180) : {wartezeiten2 = berechne_wartezeiten(startzeiten2, endzeiten2, alte_counter(2), counter(2), wartezeiten2);}
  (junction 3169) -> (junction 3209) : {timer_spuren = countOnwards(timer_spuren,1,[1 1 1 1 1 0 0]);}
  (junction 3214) -> rg3_rot_ampel4_rotgelb6 : {[autos_auf_spur6, spur6] = autos_auf_spur_generieren(spur6, gesamtZeit + timeCounter, autos_auf_spur6);}
  (junction 1180) -> (junction 1175) : {wartezeit_spur2_ges = gesamt_wartezeit_pro_spur(wartezeiten2, wartezeit_spur2_ges, alte_counter(2), counter(2));}
  (junction 1826) -> (junction 1824) : {wartezeiten6 = berechne_wartezeiten(startzeiten6, endzeiten6, alte_counter(6), counter(6), wartezeiten6);}
  rg3_rot_ampel4_rotgelb1 -> (junction 1187) : after(1,sec)
      | {timeCounter = refresher(timeCounter, 1);}
  (junction 2455) -> (junction 2463) : {wartezeiten6 = berechne_wartezeiten(startzeiten6, endzeiten6, alte_counter(6), counter(6), wartezeiten6);}
  rg3_fuss5_rot2 -> (junction 1829) : {[anz_autos6, autos_auf_spur6, counter(6), endzeiten6] = generiere_gruenphase(6, 17, autos_auf_spur6, counter(6),  (gesamtZeit + timeCounter -17), endzeiten6, startzeiten6, auslastung, autos_spur1_flag);}
  rg3_fuss5_rot5 -> (junction 2466) : {[anz_autos6, autos_auf_spur6, counter(6), endzeiten6] = generiere_gruenphase(6, 12, autos_auf_spur6, counter(6),  (gesamtZeit + timeCounter - 12), endzeiten6, startzeiten6, auslastung, autos_spur1_flag);}
  (junction 1824) -> (junction 1825) : {wartezeit_spur6_ges = gesamt_wartezeit_pro_spur(wartezeiten6, wartezeit_spur6_ges, alte_counter(6), counter(6));}
  (junction 1175) -> (junction 1195) : {gesamtwartezeit = berechne_gesamtwartezeit(wartezeit_spur1_ges, wartezeit_spur2_ges, wartezeit_spur3_ges, wartezeit_spur4_ges, wartezeit_spur5_ges, wartezeit_spur6_ges, wartezeit_spur7_ges);}
  (junction 2463) -> (junction 2464) : {wartezeit_spur6_ges = gesamt_wartezeit_pro_spur(wartezeiten6, wartezeit_spur6_ges, alte_counter(6), counter(6));}
  (junction 3209) -> rg3_fuss5_rot6 : {[autos_auf_spur6, spur6] = autos_auf_spur_generieren(spur6, gesamtZeit + timeCounter, autos_auf_spur6);}
  (junction 1187) -> ampel4_fuss5_gruen1 : {timer_spuren = countOnwards(timer_spuren,1,[1 1 1 1 1 1 1]);}
  rg3_rot_ampel4_rotgelb6 -> (junction 3204) : {[anz_autos6, autos_auf_spur6, counter(6), endzeiten6] = generiere_gruenphase(6, 10, autos_auf_spur6, counter(6),  (gesamtZeit + timeCounter - 10), endzeiten6, startzeiten6, auslastung, autos_spur1_flag);}
  (junction 1195) -> rg3_fuss5_rot1 : {gesamte_autos = berechne_gesamte_autos(counter(1), counter(2), counter(3), counter(4), counter(5), counter(6), counter(7));}
  (junction 1825) -> (junction 1807) : {gesamtwartezeit = berechne_gesamtwartezeit(wartezeit_spur1_ges, wartezeit_spur2_ges, wartezeit_spur3_ges, wartezeit_spur4_ges, wartezeit_spur5_ges, wartezeit_spur6_ges, wartezeit_spur7_ges);}
  (junction 2464) -> (junction 2465) : {gesamtwartezeit = berechne_gesamtwartezeit(wartezeit_spur1_ges, wartezeit_spur2_ges, wartezeit_spur3_ges, wartezeit_spur4_ges, wartezeit_spur5_ges, wartezeit_spur6_ges, wartezeit_spur7_ges);}
  (junction 1807) -> rg3_rot_ampel4_rotgelb3 : {gesamte_autos = berechne_gesamte_autos(counter(1), counter(2), counter(3), counter(4), counter(5), counter(6), counter(7));}
  (junction 2465) -> rg3_rot_ampel4_rotgelb5 : {gesamte_autos = berechne_gesamte_autos(counter(1), counter(2), counter(3), counter(4), counter(5), counter(6), counter(7));}
  (junction 1829) -> (junction 1828) : {wartezeiten2 = berechne_wartezeiten(startzeiten2, endzeiten2, alte_counter(2), counter(2), wartezeiten2);}
  (junction 3204) -> (junction 3205) : {wartezeiten6 = berechne_wartezeiten(startzeiten6, endzeiten6, alte_counter(6), counter(6), wartezeiten6);}
  ampel4_fuss5_gruen1 -> (junction 1167) : {[autos_auf_spur7, spur7] = autos_auf_spur_generieren(spur7, gesamtZeit + timeCounter, autos_auf_spur7);}
  (junction 2466) -> (junction 2462) : {wartezeiten2 = berechne_wartezeiten(startzeiten2, endzeiten2, alte_counter(2), counter(2), wartezeiten2);}
  rg3_fuss5_rot6 -> (junction 3220) : {[anz_autos6, autos_auf_spur6, counter(6), endzeiten6] = generiere_gruenphase(6, 10, autos_auf_spur6, counter(6),  (gesamtZeit + timeCounter -10), endzeiten6, startzeiten6, auslastung, autos_spur1_flag);}
  (junction 1828) -> (junction 1816) : {wartezeit_spur2_ges = gesamt_wartezeit_pro_spur(wartezeiten2, wartezeit_spur2_ges, alte_counter(2), counter(2));}
  (junction 1167) -> (junction 1170) : after(11,sec)
      | {timeCounter = refresher(timeCounter, 11);}
  (junction 3205) -> (junction 3217) : {wartezeit_spur6_ges = gesamt_wartezeit_pro_spur(wartezeiten6, wartezeit_spur6_ges, alte_counter(6), counter(6));}
  rg3_rot_ampel4_rotgelb3 -> (junction 1808) : after(1,sec)
      | {timeCounter = refresher(timeCounter, 1);}
  (junction 2462) -> (junction 2467) : {wartezeit_spur2_ges = gesamt_wartezeit_pro_spur(wartezeiten2, wartezeit_spur2_ges, alte_counter(2), counter(2));}
  rg3_rot_ampel4_rotgelb5 -> (junction 2468) : after(1,sec)
      | {timeCounter = refresher(timeCounter, 1);}
  (junction 1816) -> (junction 1811) : {gesamtwartezeit = berechne_gesamtwartezeit(wartezeit_spur1_ges, wartezeit_spur2_ges, wartezeit_spur3_ges, wartezeit_spur4_ges, wartezeit_spur5_ges, wartezeit_spur6_ges, wartezeit_spur7_ges);}
  (junction 1170) -> fuss5_rot : {timer_spuren = countOnwards(timer_spuren,11,[1 1 1 1 1 1 0]);}
  (junction 3217) -> (junction 3212) : {gesamtwartezeit = berechne_gesamtwartezeit(wartezeit_spur1_ges, wartezeit_spur2_ges, wartezeit_spur3_ges, wartezeit_spur4_ges, wartezeit_spur5_ges, wartezeit_spur6_ges, wartezeit_spur7_ges);}
  (junction 2467) -> (junction 2482) : {gesamtwartezeit = berechne_gesamtwartezeit(wartezeit_spur1_ges, wartezeit_spur2_ges, wartezeit_spur3_ges, wartezeit_spur4_ges, wartezeit_spur5_ges, wartezeit_spur6_ges, wartezeit_spur7_ges);}
  (junction 1808) -> ampel4_fuss5_gruen3 : {timer_spuren = countOnwards(timer_spuren,1,[1 1 1 1 1 1 1]);}
  (junction 2468) -> ampel4_fuss5_gruen5 : {timer_spuren = countOnwards(timer_spuren,1,[1 1 1 1 1 1 1]);}
  (junction 1811) -> rg3_fuss5_rot3 : {gesamte_autos = berechne_gesamte_autos(counter(1), counter(2), counter(3), counter(4), counter(5), counter(6), counter(7));}
  (junction 3212) -> rg3_rot_ampel4_rotgelb7 : {gesamte_autos = berechne_gesamte_autos(counter(1), counter(2), counter(3), counter(4), counter(5), counter(6), counter(7));}
  (junction 2482) -> rg3_fuss5_rot4 : {gesamte_autos = berechne_gesamte_autos(counter(1), counter(2), counter(3), counter(4), counter(5), counter(6), counter(7));}
  fuss5_rot -> (junction 1165)
  (junction 3220) -> (junction 3206) : {wartezeiten2 = berechne_wartezeiten(startzeiten2, endzeiten2, alte_counter(2), counter(2), wartezeiten2);}
  (junction 3206) -> (junction 3215) : {wartezeit_spur2_ges = gesamt_wartezeit_pro_spur(wartezeiten2, wartezeit_spur2_ges, alte_counter(2), counter(2));}
  ampel4_fuss5_gruen3 -> (junction 1803) : {[autos_auf_spur7, spur7] = autos_auf_spur_generieren(spur7, gesamtZeit + timeCounter, autos_auf_spur7);}
  rg3_rot_ampel4_rotgelb7 -> (junction 3207) : after(1,sec)
      | {timeCounter = refresher(timeCounter, 1);}
  ampel4_fuss5_gruen5 -> (junction 2484) : {[autos_auf_spur7, spur7] = autos_auf_spur_generieren(spur7, gesamtZeit + timeCounter, autos_auf_spur7);}
  (junction 1803) -> (junction 1802) : after(11,sec)
      | {timeCounter = refresher(timeCounter, 11);}
  (junction 3215) -> (junction 3198) : {gesamtwartezeit = berechne_gesamtwartezeit(wartezeit_spur1_ges, wartezeit_spur2_ges, wartezeit_spur3_ges, wartezeit_spur4_ges, wartezeit_spur5_ges, wartezeit_spur6_ges, wartezeit_spur7_ges);}
  (junction 2484) -> (junction 2472) : after(7,sec)
      | {timeCounter = refresher(timeCounter, 7);}
  rg3_fuss5_rot1 -> (junction 1168)
  (junction 3207) -> ampel4_fuss5_gruen7 : {timer_spuren = countOnwards(timer_spuren,1,[1 1 1 1 1 1 1]);}
  (junction 3198) -> rg3_fuss5_rot7 : {gesamte_autos = berechne_gesamte_autos(counter(1), counter(2), counter(3), counter(4), counter(5), counter(6), counter(7));}
  (junction 1802) -> fuss5_rot1 : {timer_spuren = countOnwards(timer_spuren,11,[1 1 1 1 1 1 0]);}
  (junction 2472) -> fuss5_rot2 : {timer_spuren = countOnwards(timer_spuren,7,[1 1 1 1 1 1 0]);}
  fuss5_rot1 -> (junction 1820)
  fuss5_rot2 -> (junction 2476)
  ampel4_fuss5_gruen7 -> (junction 3208) : {[autos_auf_spur7, spur7] = autos_auf_spur_generieren(spur7, gesamtZeit + timeCounter, autos_auf_spur7);}
  (junction 1165) -> (junction 1184)
  (junction 1168) -> (junction 1165)
  (junction 3208) -> (junction 3222) : after(3,sec)
      | {timeCounter = refresher(timeCounter, 3);}
  (junction 1184) -> (junction 1173) : after(2,sec)
      | {timeCounter = refresher(timeCounter, 2);}
  (junction 3222) -> fuss5_rot3 : {timer_spuren = countOnwards(timer_spuren,3,[1 1 1 1 1 1 0]);}
  rg3_fuss5_rot3 -> (junction 1801)
  (junction 1173) -> ampel4_gelb : {timer_spuren = countOnwards(timer_spuren,2,[1 1 1 1 1 1 0]);}
  rg3_fuss5_rot4 -> (junction 2474)
  fuss5_rot3 -> (junction 3194) : after(2,sec)
      | {timeCounter = refresher(timeCounter, 2);}
  ampel4_gelb -> (junction 1174) : after(3,sec)
      | {timeCounter = refresher(timeCounter, 3);}
  (junction 1174) -> (junction 1178) : {timer_spuren = countOnwards(timer_spuren,3,[1 1 1 1 1 1 0]);}
  (junction 1820) -> (junction 1800)
  (junction 1801) -> (junction 1820)
  (junction 1800) -> (junction 1804) : after(2,sec)
      | {timeCounter = refresher(timeCounter, 2);}
  (junction 2476) -> (junction 2470)
  (junction 2474) -> (junction 2476)
  (junction 2470) -> (junction 2483) : %after(1,sec)
      | %{timeCounter = refresher(timeCounter, 1);}
  (junction 1178) -> ampel4_rot : {[autos_auf_spur7, spur7] = autos_auf_spur_generieren(spur7, gesamtZeit + timeCounter, autos_auf_spur7);}
  rg3_fuss5_rot7 -> (junction 3221) : after(2,sec)
      | {timeCounter = refresher(timeCounter, 2);}
  (junction 3194) -> (junction 3210) : {timer_spuren = countOnwards(timer_spuren,2,[1 1 1 1 1 1 0]);}
  ampel4_rot -> ampel4_rot2 : {[anz_autos7, autos_auf_spur7, counter(7), endzeiten7] = generiere_gruenphase(7, 16, autos_auf_spur7, counter(7),  (gesamtZeit + timeCounter -16), endzeiten7, startzeiten7, auslastung, autos_spur1_flag);}
  (junction 1804) -> ampel4_gelb1 : {timer_spuren = countOnwards(timer_spuren,2,[1 1 1 1 1 1 0]);}
  (junction 2483) -> ampel4_gelb2 : %{timer_spuren = countOnwards(timer_spuren,1,[1 1 1 1 1 1 0]);}
  (junction 3221) -> (junction 3216) : {timer_spuren = countOnwards(timer_spuren,2,[1 1 1 1 1 1 0]);}
  ampel4_rot2 -> (junction 1181) : after(4,sec)
      | {timeCounter = refresher(timeCounter, 4);}
  (junction 3210) -> (junction 3203)
  (junction 3216) -> (junction 3210)
  (junction 3203) -> ampel4_gelb3
  ampel4_gelb1 -> (junction 1809) : after(3,sec)
      | {timeCounter = refresher(timeCounter, 3);}
  (junction 1181) -> (junction 1183) : {timer_spuren = countOnwards(timer_spuren,4,[1 1 1 1 1 1 1]);}
  ampel4_gelb2 -> (junction 2488) : after(3,sec)
      | {timeCounter = refresher(timeCounter, 3);}
  (junction 1809) -> (junction 1805) : {timer_spuren = countOnwards(timer_spuren,3,[1 1 1 1 1 1 0]);}
  (junction 1183) -> (junction 1205) : {gesamtZeit = gesamtZeit + timeCounter;}
  (junction 2488) -> (junction 2475) : {timer_spuren = countOnwards(timer_spuren,3,[1 1 1 1 1 1 0]);}
  (junction 1205) -> (junction 1207) : %{disp(startzeiten1)}
  (junction 1805) -> ampel4_rot3 : {[autos_auf_spur7, spur7] = autos_auf_spur_generieren(spur7, gesamtZeit + timeCounter, autos_auf_spur7);}
  (junction 1207) -> (junction 1215) : %{disp(endzeiten1)}
  (junction 2475) -> ampel4_rot5 : {[autos_auf_spur7, spur7] = autos_auf_spur_generieren(spur7, gesamtZeit + timeCounter, autos_auf_spur7);}
  (junction 1215) -> (junction 1212) : {wartezeiten1 = berechne_wartezeiten(startzeiten1, endzeiten1, alte_counter(1), counter(1), wartezeiten1);}
  ampel4_rot3 -> ampel4_rot4 : {[anz_autos7, autos_auf_spur7, counter(7), endzeiten7] = generiere_gruenphase(7, 16, autos_auf_spur7, counter(7),  (gesamtZeit + timeCounter -16), endzeiten7, startzeiten7, auslastung, autos_spur1_flag);}
  (junction 1212) -> (junction 1223) : {wartezeit_spur1_ges = gesamt_wartezeit_pro_spur(wartezeiten1, wartezeit_spur1_ges, alte_counter(1), counter(1));}
  ampel4_rot5 -> ampel4_rot6 : {[anz_autos7, autos_auf_spur7, counter(7), endzeiten7] = generiere_gruenphase(7, 10, autos_auf_spur7, counter(7),  (gesamtZeit + timeCounter - 10), endzeiten7, startzeiten7, auslastung, autos_spur1_flag);}
  (junction 1223) -> (junction 1214) : {wartezeiten2 = berechne_wartezeiten(startzeiten2, endzeiten2, alte_counter(2), counter(2), wartezeiten2);}
  ampel4_gelb3 -> (junction 3211) : after(3,sec)
      | {timeCounter = refresher(timeCounter, 3);}
  ampel4_rot4 -> (junction 1831) : after(4,sec)
      | {timeCounter = refresher(timeCounter, 4);}
  ampel4_rot6 -> (junction 2486) : after(4,sec)
      | {timeCounter = refresher(timeCounter, 4);}
  (junction 3211) -> (junction 3199) : {timer_spuren = countOnwards(timer_spuren,3,[1 1 1 1 1 1 0]);}
  (junction 1214) -> (junction 1198) : {wartezeit_spur2_ges = gesamt_wartezeit_pro_spur(wartezeiten2, wartezeit_spur2_ges, alte_counter(2), counter(2));}
  (junction 1831) -> (junction 1817) : {timer_spuren = countOnwards(timer_spuren,4,[1 1 1 1 1 1 1]);}
  (junction 3199) -> ampel4_rot7 : {[autos_auf_spur7, spur7] = autos_auf_spur_generieren(spur7, gesamtZeit + timeCounter, autos_auf_spur7);}
  (junction 2486) -> (junction 2487) : {timer_spuren = countOnwards(timer_spuren,4,[1 1 1 1 1 1 1]);}
  (junction 1817) -> (junction 1806) : {gesamtZeit = gesamtZeit + timeCounter;}
  (junction 1198) -> (junction 1222) : {wartezeiten3 = berechne_wartezeiten(startzeiten3, endzeiten3, alte_counter(3), counter(3), wartezeiten3);}
  (junction 2487) -> (junction 2473) : {gesamtZeit = gesamtZeit + timeCounter;}
  (junction 1806) -> (junction 1810) : %{disp(startzeiten1)}
  (junction 2473) -> (junction 2485) : %{disp(startzeiten1)}
  ampel4_rot7 -> ampel4_rot8 : {[anz_autos7, autos_auf_spur7, counter(7), endzeiten7] = generiere_gruenphase(7, 10, autos_auf_spur7, counter(7),  (gesamtZeit + timeCounter -10), endzeiten7, startzeiten7, auslastung, autos_spur1_flag);}
  (junction 1810) -> (junction 1812) : %{disp(endzeiten1)}
  (junction 1222) -> (junction 1209) : {wartezeit_spur3_ges = gesamt_wartezeit_pro_spur(wartezeiten3, wartezeit_spur3_ges, alte_counter(3), counter(3));}
  (junction 2485) -> (junction 2471) : %{disp(endzeiten1)}
  (junction 1812) -> (junction 1814) : {wartezeiten1 = berechne_wartezeiten(startzeiten1, endzeiten1, alte_counter(1), counter(1), wartezeiten1);}
  (junction 2471) -> (junction 2477) : {wartezeiten1 = berechne_wartezeiten(startzeiten1, endzeiten1, alte_counter(1), counter(1), wartezeiten1);}
  (junction 1209) -> (junction 1206) : {wartezeiten4 = berechne_wartezeiten(startzeiten4, endzeiten4, alte_counter(4), counter(4), wartezeiten4);}
  (junction 1814) -> (junction 1827) : {wartezeit_spur1_ges = gesamt_wartezeit_pro_spur(wartezeiten1, wartezeit_spur1_ges, alte_counter(1), counter(1));}
  ampel4_rot8 -> (junction 3193) : after(4,sec)
      | {timeCounter = refresher(timeCounter, 4);}
  (junction 2477) -> (junction 2478) : {wartezeit_spur1_ges = gesamt_wartezeit_pro_spur(wartezeiten1, wartezeit_spur1_ges, alte_counter(1), counter(1));}
  (junction 1206) -> (junction 1213) : {wartezeit_spur4_ges = gesamt_wartezeit_pro_spur(wartezeiten4, wartezeit_spur4_ges, alte_counter(4), counter(4));}
  (junction 1827) -> (junction 1813) : {wartezeiten2 = berechne_wartezeiten(startzeiten2, endzeiten2, alte_counter(2), counter(2), wartezeiten2);}
  (junction 2478) -> (junction 2479) : {wartezeiten2 = berechne_wartezeiten(startzeiten2, endzeiten2, alte_counter(2), counter(2), wartezeiten2);}
  (junction 3193) -> (junction 3201) : {timer_spuren = countOnwards(timer_spuren,4,[1 1 1 1 1 1 1]);}
  (junction 1213) -> (junction 1200) : {wartezeiten5 = berechne_wartezeiten(startzeiten5, endzeiten5, alte_counter(5), counter(5), wartezeiten5);}
  (junction 3201) -> (junction 3218) : {gesamtZeit = gesamtZeit + timeCounter;}
  (junction 1813) -> (junction 1815) : {wartezeit_spur2_ges = gesamt_wartezeit_pro_spur(wartezeiten2, wartezeit_spur2_ges, alte_counter(2), counter(2));}
  (junction 1200) -> (junction 1220) : {wartezeit_spur5_ges = gesamt_wartezeit_pro_spur(wartezeiten5, wartezeit_spur5_ges, alte_counter(5), counter(5));}
  (junction 3218) -> (junction 3191) : %{disp(startzeiten1)}
  (junction 2479) -> (junction 2489) : {wartezeit_spur2_ges = gesamt_wartezeit_pro_spur(wartezeiten2, wartezeit_spur2_ges, alte_counter(2), counter(2));}
  (junction 3191) -> (junction 3213) : %{disp(endzeiten1)}
  (junction 1220) -> (junction 1219) : {wartezeiten6 = berechne_wartezeiten(startzeiten6, endzeiten6, alte_counter(6), counter(6), wartezeiten6);}
  (junction 1815) -> (junction 1818) : {wartezeiten3 = berechne_wartezeiten(startzeiten3, endzeiten3, alte_counter(3), counter(3), wartezeiten3);}
  (junction 3213) -> (junction 3196) : {wartezeiten1 = berechne_wartezeiten(startzeiten1, endzeiten1, alte_counter(1), counter(1), wartezeiten1);}
  (junction 2489) -> (junction 2469) : {wartezeiten3 = berechne_wartezeiten(startzeiten3, endzeiten3, alte_counter(3), counter(3), wartezeiten3);}
  (junction 1219) -> (junction 1217) : {wartezeit_spur6_ges = gesamt_wartezeit_pro_spur(wartezeiten6, wartezeit_spur6_ges, alte_counter(6), counter(6));}
  (junction 1818) -> (junction 1830) : {wartezeit_spur3_ges = gesamt_wartezeit_pro_spur(wartezeiten3, wartezeit_spur3_ges, alte_counter(3), counter(3));}
  (junction 3196) -> (junction 3192) : {wartezeit_spur1_ges = gesamt_wartezeit_pro_spur(wartezeiten1, wartezeit_spur1_ges, alte_counter(1), counter(1));}
  (junction 1217) -> (junction 1216) : %{disp(startzeiten7)}
  (junction 2469) -> (junction 2480) : {wartezeit_spur3_ges = gesamt_wartezeit_pro_spur(wartezeiten3, wartezeit_spur3_ges, alte_counter(3), counter(3));}
  (junction 3192) -> (junction 3200) : {wartezeiten2 = berechne_wartezeiten(startzeiten2, endzeiten2, alte_counter(2), counter(2), wartezeiten2);}
  (junction 1830) -> (junction 1819) : {wartezeiten4 = berechne_wartezeiten(startzeiten4, endzeiten4, alte_counter(4), counter(4), wartezeiten4);}
  (junction 1216) -> (junction 1208) : %{disp(endzeiten7)}
  (junction 2480) -> (junction 2481) : {wartezeiten4 = berechne_wartezeiten(startzeiten4, endzeiten4, alte_counter(4), counter(4), wartezeiten4);}
  (junction 3200) -> (junction 3219) : {wartezeit_spur2_ges = gesamt_wartezeit_pro_spur(wartezeiten2, wartezeit_spur2_ges, alte_counter(2), counter(2));}
  (junction 1819) -> (junction 1821) : {wartezeit_spur4_ges = gesamt_wartezeit_pro_spur(wartezeiten4, wartezeit_spur4_ges, alte_counter(4), counter(4));}
  (junction 2481) -> (junction 2511) : {wartezeit_spur4_ges = gesamt_wartezeit_pro_spur(wartezeiten4, wartezeit_spur4_ges, alte_counter(4), counter(4));}
  (junction 1821) -> (junction 1822) : {wartezeiten5 = berechne_wartezeiten(startzeiten5, endzeiten5, alte_counter(5), counter(5), wartezeiten5);}
  (junction 1208) -> (junction 1199) : {wartezeiten7 = berechne_wartezeiten(startzeiten7, endzeiten7, alte_counter(7), counter(7), wartezeiten7);}
  (junction 2511) -> (junction 2522) : {wartezeiten5 = berechne_wartezeiten(startzeiten5, endzeiten5, alte_counter(5), counter(5), wartezeiten5);}
  (junction 3219) -> (junction 3195) : {wartezeiten3 = berechne_wartezeiten(startzeiten3, endzeiten3, alte_counter(3), counter(3), wartezeiten3);}
  (junction 1822) -> (junction 1823) : {wartezeit_spur5_ges = gesamt_wartezeit_pro_spur(wartezeiten5, wartezeit_spur5_ges, alte_counter(5), counter(5));}
  (junction 2522) -> (junction 2495) : {wartezeit_spur5_ges = gesamt_wartezeit_pro_spur(wartezeiten5, wartezeit_spur5_ges, alte_counter(5), counter(5));}
  (junction 1823) -> (junction 1832) : {wartezeiten6 = berechne_wartezeiten(startzeiten6, endzeiten6, alte_counter(6), counter(6), wartezeiten6);}
  (junction 3195) -> (junction 3197) : {wartezeit_spur3_ges = gesamt_wartezeit_pro_spur(wartezeiten3, wartezeit_spur3_ges, alte_counter(3), counter(3));}
  (junction 1199) -> (junction 1196) : {wartezeit_spur7_ges = gesamt_wartezeit_pro_spur(wartezeiten7, wartezeit_spur7_ges, alte_counter(7), counter(7));}
  (junction 2495) -> (junction 2512) : {wartezeiten6 = berechne_wartezeiten(startzeiten6, endzeiten6, alte_counter(6), counter(6), wartezeiten6);}
  (junction 1832) -> (junction 1837) : {wartezeit_spur6_ges = gesamt_wartezeit_pro_spur(wartezeiten6, wartezeit_spur6_ges, alte_counter(6), counter(6));}
  (junction 2512) -> (junction 2491) : {wartezeit_spur6_ges = gesamt_wartezeit_pro_spur(wartezeiten6, wartezeit_spur6_ges, alte_counter(6), counter(6));}
  (junction 3197) -> (junction 3202) : {wartezeiten4 = berechne_wartezeiten(startzeiten4, endzeiten4, alte_counter(4), counter(4), wartezeiten4);}
  (junction 1837) -> (junction 1833) : %{disp(startzeiten7)}
  (junction 2491) -> (junction 2499) : %{disp(startzeiten7)}
  (junction 3202) -> (junction 3235) : {wartezeit_spur4_ges = gesamt_wartezeit_pro_spur(wartezeiten4, wartezeit_spur4_ges, alte_counter(4), counter(4));}
  (junction 1196) -> (junction 1218) : {gesamtwartezeit = berechne_gesamtwartezeit(wartezeit_spur1_ges, wartezeit_spur2_ges, wartezeit_spur3_ges, wartezeit_spur4_ges, wartezeit_spur5_ges, wartezeit_spur6_ges, wartezeit_spur7_ges)}
  (junction 1833) -> (junction 1835) : %{disp(endzeiten7)}
  (junction 3235) -> (junction 3229) : {wartezeiten5 = berechne_wartezeiten(startzeiten5, endzeiten5, alte_counter(5), counter(5), wartezeiten5);}
  (junction 2499) -> (junction 2497) : %{disp(endzeiten7)}
  (junction 3229) -> (junction 3232) : {wartezeit_spur5_ges = gesamt_wartezeit_pro_spur(wartezeiten5, wartezeit_spur5_ges, alte_counter(5), counter(5));}
  (junction 1835) -> (junction 1838) : {wartezeiten7 = berechne_wartezeiten(startzeiten7, endzeiten7, alte_counter(7), counter(7), wartezeiten7);}
  (junction 3232) -> (junction 3234) : {wartezeiten6 = berechne_wartezeiten(startzeiten6, endzeiten6, alte_counter(6), counter(6), wartezeiten6);}
  (junction 2497) -> (junction 2494) : {wartezeiten7 = berechne_wartezeiten(startzeiten7, endzeiten7, alte_counter(7), counter(7), wartezeiten7);}
  (junction 1218) -> (junction 1201) : {gesamte_autos = berechne_gesamte_autos(counter(1), counter(2), counter(3), counter(4), counter(5), counter(6), counter(7))}
  (junction 3234) -> (junction 3223) : {wartezeit_spur6_ges = gesamt_wartezeit_pro_spur(wartezeiten6, wartezeit_spur6_ges, alte_counter(6), counter(6));}
  (junction 1838) -> (junction 1834) : {wartezeit_spur7_ges = gesamt_wartezeit_pro_spur(wartezeiten7, wartezeit_spur7_ges, alte_counter(7), counter(7));}
  (junction 3223) -> (junction 3230) : %{disp(startzeiten7)}
  (junction 2494) -> (junction 2525) : {wartezeit_spur7_ges = gesamt_wartezeit_pro_spur(wartezeiten7, wartezeit_spur7_ges, alte_counter(7), counter(7));}
  (junction 1201) -> (junction 1202) : {runden_ueberquerte_autos = counter(1) - alte_counter(1) + counter(2) - alte_counter(2) + counter(3) - alte_counter(3) + counter(4) - alte_counter(4) + counter(5) - alte_counter(5) + counter(6) - alte_counter(6) + counter(7) - alte_counter(7);}
  (junction 3230) -> (junction 3227) : %{disp(endzeiten7)}
  (junction 1202) -> (junction 1221) : {krit1 = runden_ueberquerte_autos / timeCounter;}
  (junction 1834) -> (junction 1836) : {gesamtwartezeit = berechne_gesamtwartezeit(wartezeit_spur1_ges, wartezeit_spur2_ges, wartezeit_spur3_ges, wartezeit_spur4_ges, wartezeit_spur5_ges, wartezeit_spur6_ges, wartezeit_spur7_ges)}
  (junction 2525) -> (junction 2514) : {gesamtwartezeit = berechne_gesamtwartezeit(wartezeit_spur1_ges, wartezeit_spur2_ges, wartezeit_spur3_ges, wartezeit_spur4_ges, wartezeit_spur5_ges, wartezeit_spur6_ges, wartezeit_spur7_ges)}
  (junction 3227) -> (junction 3224) : {wartezeiten7 = berechne_wartezeiten(startzeiten7, endzeiten7, alte_counter(7), counter(7), wartezeiten7);}
  (junction 1221) -> (junction 1203) : {krit2 = gesamte_autos / (gesamtZeit + timeCounter);}
  (junction 3224) -> (junction 3233) : {wartezeit_spur7_ges = gesamt_wartezeit_pro_spur(wartezeiten7, wartezeit_spur7_ges, alte_counter(7), counter(7));}
  (junction 1836) -> (junction 1441) : {gesamte_autos = berechne_gesamte_autos(counter(1), counter(2), counter(3), counter(4), counter(5), counter(6), counter(7))}
  (junction 2514) -> (junction 2496) : {gesamte_autos = berechne_gesamte_autos(counter(1), counter(2), counter(3), counter(4), counter(5), counter(6), counter(7))}
  (junction 1203) -> (junction 1204) : {krit3 = gesamtwartezeit / gesamte_autos;}
  (junction 1441) -> (junction 1437) : {runden_ueberquerte_autos = counter(1) - alte_counter(1) + counter(2) - alte_counter(2) + counter(3) - alte_counter(3) + counter(4) - alte_counter(4) + counter(5) - alte_counter(5) + counter(6) - alte_counter(6) + counter(7) - alte_counter(7);}
  (junction 2496) -> (junction 2518) : {runden_ueberquerte_autos = counter(1) - alte_counter(1) + counter(2) - alte_counter(2) + counter(3) - alte_counter(3) + counter(4) - alte_counter(4) + counter(5) - alte_counter(5) + counter(6) - alte_counter(6) + counter(7) - alte_counter(7);}
  (junction 3233) -> (junction 3226) : {gesamtwartezeit = berechne_gesamtwartezeit(wartezeit_spur1_ges, wartezeit_spur2_ges, wartezeit_spur3_ges, wartezeit_spur4_ges, wartezeit_spur5_ges, wartezeit_spur6_ges, wartezeit_spur7_ges)}
  (junction 1437) -> (junction 1433) : {krit1 = runden_ueberquerte_autos / timeCounter;}
  (junction 2518) -> (junction 2513) : {krit1 = runden_ueberquerte_autos / timeCounter;}
  (junction 1204) -> (junction 3349)
  (junction 3226) -> (junction 3231) : {gesamte_autos = berechne_gesamte_autos(counter(1), counter(2), counter(3), counter(4), counter(5), counter(6), counter(7))}
  (junction 1433) -> (junction 1434) : {krit2 = gesamte_autos / (gesamtZeit + timeCounter);}
  (junction 2513) -> (junction 2516) : {krit2 = gesamte_autos / (gesamtZeit + timeCounter);}
  (junction 3231) -> (junction 3237) : {runden_ueberquerte_autos = counter(1) - alte_counter(1) + counter(2) - alte_counter(2) + counter(3) - alte_counter(3) + counter(4) - alte_counter(4) + counter(5) - alte_counter(5) + counter(6) - alte_counter(6) + counter(7) - alte_counter(7);}
  (junction 1434) -> (junction 1478) : {krit3 = gesamtwartezeit / gesamte_autos;}
  (junction 2516) -> (junction 2524) : {krit3 = gesamtwartezeit / gesamte_autos;}
  (junction 3237) -> (junction 3236) : {krit1 = runden_ueberquerte_autos / timeCounter;}
  (junction 2524) -> (junction 3343)
  (junction 1478) -> (junction 3346)
  (junction 3236) -> (junction 3225) : {krit2 = gesamte_autos / (gesamtZeit + timeCounter);}
  (junction 3225) -> (junction 3228) : {krit3 = gesamtwartezeit / gesamte_autos;}
  (junction 3228) -> (junction 3338)
  (junction 3338) -> (junction 179)
  (junction 3343) -> (junction 3338)
  (junction 3346) -> (junction 3343)
  (junction 3349) -> (junction 3346)
  data: autos_neu_fkt function_output; N_fkt function_input; zeit_abstand_fkt function_input; auslastung_fkt function_input; autos_fkt function_input; spur1fkt function_output; spur2fkt function_output; spur3fkt function_output; spur4fkt function_output; spur5fkt function_output; spur6fkt function_output; spur7fkt function_output; N_fkt function_input; spur_autos function_input; timer function_input; autos_auf_spur_fkt function_input; autos_auf_spur_fkt function_output; spur_autos function_output; spur function_input; laenge function_input; autos_auf_spur_u function_input; counter_alt function_input; start_timer_fkt function_input; endzeiten function_input; anz_autos_fkt function_output; autos_auf_spur_fkt function_output; counter_neu_fkt function_output; endzeiten function_output; startzeiten_fkt function_input; auslastung_fkt function_input; autos_spur1_flag_fkt function_input; auslastung_fkt function_input; zeit_abstand_fkt function_output; time function_input; timeElapsed function_input; spuren function_input; count_spur function_output; timer function_output; timer function_output; startTime function_input; timeElapsed function_input; startzeiten_fkt function_input; endzeiten_fkt function_input; alter_counter_fkt function_input; counter_fkt function_input; wartezeiten_fkt_u function_input; wartezeiten_fkt function_output; wartezeit_fkt function_input; spur_wartezeit_u function_input; counter_alt_fkt function_input; spur_wartezeit_fkt function_output double; counter_fkt function_input; ges_wartezeit1_fkt function_input; ges_wartezeit2_fkt function_input; ges_wartezeit3_fkt function_input; ges_wartezeit4_fkt function_input; ges_wartezeit5_fkt function_input; ges_wartezeit6_fkt function_input; ges_wartezeit7_fkt function_input; gesamtwartezeit_fkt function_output; counter1_fkt function_input; counter2_fkt function_input; counter3_fkt function_input; counter4_fkt function_input; counter5_fkt function_input; counter6_fkt function_input; counter7_fkt function_input; gesamte_autos_fkt function_output; rot1_l output; gelb1_l output; gruen1_l output; rot1_rg output; gelb1_rg output; gruen1_rg output; rot2 output; gelb2 output; gruen2 output; rot3_l output; gelb3_l output; gruen3_l output; rot3_rg output; gelb3_rg output; gruen3_rg output; rot4 output; gelb4 output; gruen4 output; rot5 output; gruen5 output; rot6 output; gruen6 output; rot7 output; gruen7 output; rot8 output; gruen8 output; autos_auf_spur1 output; timer_spuren local; anz_autos1 local; anz_autos2 local; anz_autos3 local; anz_autos4 local; anz_autos5 local; anz_autos6 local; anz_autos7 local; alte_counter local; counter local; endzeiten1 local; endzeiten2 local; endzeiten3 local; endzeiten4 local; endzeiten5 local; endzeiten6 local; endzeiten7 local; spur1 local; spur2 local; spur3 local; spur4 local; spur5 local; spur6 local; spur7 local; startzeiten7 local; wartezeiten1 local; startzeiten1 local; startzeiten2 local; startzeiten3 local; startzeiten4 local; startzeiten5 local; startzeiten6 local; wartezeiten2 local; wartezeiten3 local; wartezeiten4 local; wartezeiten5 local; wartezeiten6 local; wartezeiten7 local; autos_auf_spur2 output; autos_auf_spur3 output; autos_auf_spur4 output; autos_auf_spur5 output; autos_auf_spur6 output; autos_auf_spur7 output; wartezeit_spur1_ges output; wartezeit_spur2_ges output; wartezeit_spur3_ges output; wartezeit_spur4_ges output; wartezeit_spur5_ges output; wartezeit_spur6_ges output; wartezeit_spur7_ges output; gesamtwartezeit output; timeCounter output; gesamtZeit output; alle_autos_neu local; N constant double =10000; auslastung input; zeit_abstand local; gesamte_autos output; krit1 output; krit2 output; runden_ueberquerte_autos local; krit3 output; autos_spur1_flag local
  function autos_neu_fkt = generiere_autos_neu(N_fkt, zeit_abstand_fkt, auslastung_fkt):
    | function autos_neu_fkt = generiere_autos_neu(N_fkt, zeit_abstand_fkt, auslastung_fkt)
    |     zeiten_fkt = zeros(1,N_fkt); %Platzhalter für Spawnzeiten
    |     for i=1:N
    |         zeiten_fkt(i) = zeit_abstand_fkt * i + randn();
    |         if zeiten_fkt(i) < 0
    |             zeiten_fkt(i) = 0
    |         end
    |     end
    | 	
    |     switch (auslastung_fkt)
    |         case 1
    |             wahrscheinlichkeiten = [0.12, 0.20, 0.12, 0.20, 0.12, 0.12, 0.12];
    |         case 2
    |             wahrscheinlichkeiten = [0.08, 0.28, 0.08, 0.28, 0.08, 0.08, 0.12];
    |         case 3
    |             wahrscheinlichkeiten = [0.06, 0.32, 0.085, 0.265, 0.07, 0.12, 0.13];
    |         case 4
    |             wahrscheinlichkeiten = [0.05, 0.2525, 0.14, 0.3175, 0.055, 0.095, 0.14];
    |         case 5
    |             wahrscheinlichkeiten = [0.05, 0.27, 0.135, 0.305, 0.06, 0.095, 0.135];
    |         otherwise
    |             wahrscheinlichkeiten = [0.06, 0.32, 0.07, 0.26, 0.09, 0.12, 0.13];
    |     end
    |     
    |     spuren_werte = [1, 2, 3, 4, 5, 6, 7]; % Die entsprechenden Werte
    | 
    |     kumulative_wahrscheinlichkeiten = cumsum(wahrscheinlichkeiten);
    | 
    |     zufaellige_nummer = rand(1, N_fkt);
    |     spuren = zeros(1, N_fkt); % Platzhalter für die Spuren
    | 
    |     % Werte basierend auf Wahrscheinlichkeiten zuweisen
    |     for i = 1:N_fkt
    |         spuren(i) = spuren_werte(find(zufaellige_nummer(i) <= kumulative_wahrscheinlichkeiten, 1));
    |     end
    | 
    |     zeiten_fkt = sort(zeiten_fkt);
    | 
    |     autos_neu_fkt = [spuren; zeiten_fkt];
    | end
  function [spur1fkt, spur2fkt, spur3fkt, spur4fkt, spur5fkt, spur6fkt, spur7fkt] = spuren_aus_autos(autos_fkt, N_fkt):
    | function [spur1fkt, spur2fkt, spur3fkt, spur4fkt, spur5fkt, spur6fkt, spur7fkt] = spuren_aus_autos(autos_fkt, N_fkt)
    |     counter1 = 1; counter2 = 1; counter3 = 1; counter4 = 1; counter5 = 1; counter6 = 1; counter7 = 1;
    |     spur1fkt = zeros(1,N_fkt/2);
    |     spur2fkt = zeros(1,N_fkt/2);
    |     spur3fkt = zeros(1,N_fkt/2);
    |     spur4fkt = zeros(1,N_fkt/2);
    |     spur5fkt = zeros(1,N_fkt/2);
    |     spur6fkt = zeros(1,N_fkt/2);
    |     spur7fkt = zeros(1,N_fkt/2);
    |     for i = 1:length(autos_fkt)
    |         switch(autos_fkt(1,i))
    |             case 1
    |                 %spur1fkt
    |                 %spur1fkt(counter1)
    |                 %autos_fkt
    |                 %autos_fkt(2,i)
    |                 spur1fkt(counter1) = autos_fkt(2,i);
    |                 counter1 = counter1 + 1;
    |             case 2
    |                 %spur2fkt
    |                 %spur2fkt(counter2)
    |                 %autos_fkt
    |                 %autos_fkt(2,i)
    |                 spur2fkt(counter2) = autos_fkt(2,i);
    |                 counter2 = counter2 + 1;
    |             case 3
    |                 spur3fkt(counter3) = autos_fkt(2,i);
    |                 counter3 = counter3 + 1;
    |             case 4
    |                 spur4fkt(counter4) = autos_fkt(2,i);
    |                 counter4 = counter4 + 1;
    |             case 5
    |                 spur5fkt(counter5) = autos_fkt(2,i);
    |                 counter5 = counter5 + 1;
    |             case 6
    |                 spur6fkt(counter6) = autos_fkt(2,i);
    |                 counter6 = counter6 + 1;
    |             case 7
    |                 spur7fkt(counter7) = autos_fkt(2,i);
